simulink model "h16k_ver110_1080"  (R2012b)
settings: Solver=VariableStepDiscrete  SolverMode=SingleTasking  StartTime=0.0  StopTime=128000  RelTol=1e-3
undefined symbols (not defined in the file or in its folder): sfp
libraries: xbsIndex_r4 x3384, dspsigops x32, casper_library_misc x23, monroe_library x8, simulink x7, xps_library x6
(part 1 of 28)
settings Model: Creator=mwagner  LastModifiedBy=ptcs
settings DataIOCC: SignalLoggingSaveFormat=ModelDataLogs
settings OptimizationCC: InlineParams=on
settings DebuggingCC: FcnCallInpInsideContextMsg=UseLocalSettings  StrictBusMsg=Warning
settings GRTTargetCC: CombineOutputUpdateFcns=off  GRTInterface=on

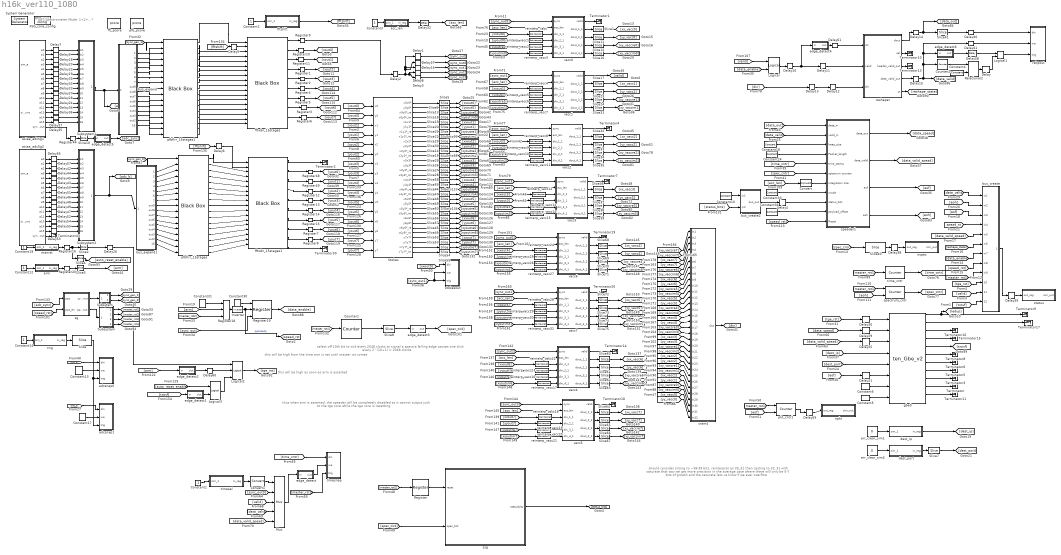
== system h16k_ver110_1080 ==
  note: GBT Spectrometer
      | Mode: 1+2+...?
  note: this will be high from the time arm is set until master rst comes
  note: this will be high as soon as arm is asserted
  note: thus when arm is asserted, the speader will be completely disabled so it cannot output junk to the tge core while the tge core is resetting
  note: should consider slicing to ~38-39 bits, reinterpret as 39_31 then casting to  32_31 with saturate
      | that way we get more precision in the average case where there will only be 5-7 bits of growth
      | and the saturate lets us know if we ever overflow
  note: select off 10th bit to tick every 2048 clocks to signal a spectra
      | falling edge causes one click every 2^(10+1) = 2048 clocks
  " System Generator" : xbsIndex_r4/ System Generator  Tag=genX  xilinxfamily=virtex6  part=xc6vsx475t  speed=-1  package=ff1759  synthesis_tool=XST  clock_wrapper=Clock Enables  directory=./h16k_ver110_1080/sysgen  proj_type=Project Navigator  Synth_file=XST Defaults  Impl_file=ISE Defaults  testbench=off  simulink_period=1  sysclk_period=7.4074  dcm_input_clock_period=100  incr_netlist=off  trim_vbits=Everywhere in SubSystem  dbl_ovrd=According to Block Masks  core_generation=According to Block Masks  run_coregen=off  deprecated_control=off  eval_field=0  block_type=sysgen
      settings: block_version=10.1.3
  Constant{1..3,12,14,19} (6 alike) : Constant
  Constant10 : xbsIndex_r4/Constant  const=0  gui_display_data_type=Fixed-point  arith_type=Unsigned  n_bits=36  bin_pt=0  preci_type=Single  exp_width=8  frac_width=24  explicit_period=on  period=1  equ=P=C  opselect=C  inp2=PCIN>>17  opr=+  inp1=P  carry=CIN  dbl_ovrd=off  block_type=constant
  Constant13 : xbsIndex_r4/Constant  const=1  gui_display_data_type=Boolean  arith_type=Boolean  n_bits=32  bin_pt=0  preci_type=Single  exp_width=8  frac_width=24  explicit_period=on  period=1  equ=P=C  opselect=C  inp2=PCIN>>17  opr=+  inp1=P  carry=CIN  dbl_ovrd=off  block_type=constant
      settings: block_version=11.4
  Constant17 : xbsIndex_r4/Constant  const=1  gui_display_data_type=Boolean  arith_type=Boolean  n_bits=32  bin_pt=0  preci_type=Single  exp_width=8  frac_width=24  explicit_period=on  period=1  equ=P=C  opselect=C  inp2=PCIN>>17  opr=+  inp1=P  carry=CIN  dbl_ovrd=off  block_type=constant
      settings: block_version=11.4
  Constant18 : xbsIndex_r4/Constant  const=262144+8*6  gui_display_data_type=Fixed-point  arith_type=Unsigned  n_bits=40  bin_pt=0  preci_type=Single  exp_width=8  frac_width=24  explicit_period=on  period=1  equ=P=C  opselect=C  inp2=PCIN>>17  opr=+  inp1=P  carry=CIN  dbl_ovrd=off  block_type=constant
  Constant24 : xbsIndex_r4/Constant  const=8192  gui_display_data_type=Fixed-point  arith_type=Unsigned  n_bits=40  bin_pt=0  preci_type=Single  exp_width=8  frac_width=24  explicit_period=on  period=1  equ=P=C  opselect=C  inp2=PCIN>>17  opr=+  inp1=P  carry=CIN  dbl_ovrd=off  block_type=constant
  Constant30 : xbsIndex_r4/Constant  const=1  gui_display_data_type=Fixed-point  arith_type=Boolean  n_bits=16  bin_pt=0  preci_type=Single  exp_width=8  frac_width=24  explicit_period=on  period=1  equ=P=C  opselect=C  inp2=PCIN>>17  opr=+  inp1=P  carry=CIN  dbl_ovrd=off  block_type=constant
      settings: block_version=11.4
  Constant31 : xbsIndex_r4/Constant  const=1  gui_display_data_type=Fixed-point  arith_type=Boolean  n_bits=16  bin_pt=0  preci_type=Single  exp_width=8  frac_width=24  explicit_period=on  period=1  equ=P=C  opselect=C  inp2=PCIN>>17  opr=+  inp1=P  carry=CIN  dbl_ovrd=off  block_type=constant
      settings: block_version=11.4
  Constant33 : xbsIndex_r4/Constant  const=1  gui_display_data_type=Fixed-point  arith_type=Unsigned  n_bits=40  bin_pt=0  preci_type=Single  exp_width=8  frac_width=24  explicit_period=on  period=1  equ=P=C  opselect=C  inp2=PCIN>>17  opr=+  inp1=P  carry=CIN  dbl_ovrd=off  block_type=constant
  Constant34 : xbsIndex_r4/Constant  const=0  gui_display_data_type=Fixed-point  arith_type=Unsigned  n_bits=40  bin_pt=0  preci_type=Single  exp_width=8  frac_width=24  explicit_period=on  period=1  equ=P=C  opselect=C  inp2=PCIN>>17  opr=+  inp1=P  carry=CIN  dbl_ovrd=off  block_type=constant
  Constant4 : xbsIndex_r4/Constant  const=65535  gui_display_data_type=Fixed-point  arith_type=Unsigned  n_bits=16  bin_pt=0  preci_type=Single  exp_width=8  frac_width=24  explicit_period=on  period=1  equ=P=C  opselect=C  inp2=PCIN>>17  opr=+  inp1=P  carry=CIN  dbl_ovrd=off  block_type=constant
  Constant5 : xbsIndex_r4/Constant  const=1  gui_display_data_type=Boolean  arith_type=Boolean  n_bits=1  bin_pt=0  preci_type=Single  exp_width=8  frac_width=24  explicit_period=on  period=1  equ=P=C  opselect=C  inp2=PCIN>>17  opr=+  inp1=P  carry=CIN  dbl_ovrd=off  block_type=constant
  Constant6 : xbsIndex_r4/Constant  const=1  gui_display_data_type=Boolean  arith_type=Boolean  n_bits=1  bin_pt=0  preci_type=Single  exp_width=8  frac_width=24  explicit_period=on  period=1  equ=P=C  opselect=C  inp2=PCIN>>17  opr=+  inp1=P  carry=CIN  dbl_ovrd=off  block_type=constant
  Convert : xbsIndex_r4/Convert  gui_display_data_type=Fixed-point  arith_type=Unsigned  n_bits=40  bin_pt=0  float_type=Single  exp_bits=8  fraction_bits=24  quantization=Truncate  overflow=Wrap  en=off  latency=0  dbl_ovrd=off  pipeline=off  block_type=convert
      settings: block_version=11.4
  Convert1 : xbsIndex_r4/Convert  gui_display_data_type=Fixed-point  arith_type=Unsigned  n_bits=2  bin_pt=0  float_type=Single  exp_bits=8  fraction_bits=24  quantization=Truncate  overflow=Wrap  en=off  latency=1  dbl_ovrd=off  pipeline=off  block_type=convert
  Counter1 : xbsIndex_r4/Counter  cnt_type=Free Running  cnt_to=Inf  operation=Up  start_count=0  cnt_by_val=1  arith_type=Unsigned  n_bits=48  bin_pt=0  load_pin=off  rst=on  en=off  explicit_period=on  period=1  dbl_ovrd=off  use_behavioral_HDL=off  implementation=DSP48  block_type=counter
      settings: block_version=11.3
  Counter2 : xbsIndex_r4/Counter  cnt_type=Free Running  cnt_to=Inf  operation=Down  start_count=65535  cnt_by_val=1  arith_type=Unsigned  n_bits=16  bin_pt=0  load_pin=off  rst=off  en=on  explicit_period=on  period=1  dbl_ovrd=off  use_behavioral_HDL=off  implementation=Fabric  block_type=counter
  Delay{,1,3,5..6,8,16..17,32} (9 alike) : xbsIndex_r4/Delay  rst=off  infoeditControl=Selection of Reset will increase slice count due to use of real FFs and instead of SRLs  en=off  latency=1  dbl_ovrd=off  reg_retiming=off  block_type=delay
      Delay1 settings: block_version=11.4
      Delay16 settings: block_version=11.4
      Delay17 settings: block_version=11.4
      Delay3 settings: block_version=11.4
      Delay32 settings: block_version=11.4
      Delay5 settings: block_version=11.4
      Delay6 settings: block_version=11.4
      Delay8 settings: block_version=11.4
  Delay{10..13,58} (5 alike) : xbsIndex_r4/Delay  rst=off  infoeditControl=Selection of Reset will increase slice count due to use of real FFs and instead of SRLs  en=off  latency=2  dbl_ovrd=off  reg_retiming=off  block_type=delay
  Delay{14..15,40..41} (4 alike) : xbsIndex_r4/Delay  rst=off  infoeditControl=Selection of Reset will increase slice count due to use of real FFs and instead of SRLs  en=off  latency=4  dbl_ovrd=off  reg_retiming=on  block_type=delay
  Delay{4,7,9,18..25,27..31,33..39,42..57,59} (40 alike) : xbsIndex_r4/Delay  rst=off  infoeditControl=Selection of Reset will increase slice count due to use of real FFs and instead of SRLs  en=off  latency=1  dbl_ovrd=off  reg_retiming=on  block_type=delay
      Delay18 settings: block_version=11.4
      Delay19 settings: block_version=11.4
      Delay20 settings: block_version=11.4
      Delay22 settings: block_version=11.4
      Delay23 settings: block_version=11.4
      Delay24 settings: block_version=11.4
      Delay27 settings: block_version=11.4
      Delay28 settings: block_version=11.4
      Delay31 settings: block_version=11.4
      Delay33 settings: block_version=11.4
      Delay34 settings: block_version=11.4
      Delay35 settings: block_version=11.4
      Delay36 settings: block_version=11.4
      Delay37 settings: block_version=11.4
      Delay42 settings: block_version=11.4
      Delay43 settings: block_version=11.4
      Delay44 settings: block_version=11.4
      Delay45 settings: block_version=11.4
      Delay46 settings: block_version=11.4
      Delay47 settings: block_version=11.4
      Delay48 settings: block_version=11.4
      Delay49 settings: block_version=11.4
      Delay50 settings: block_version=11.4
      Delay51 settings: block_version=11.4
      Delay52 settings: block_version=11.4
      Delay53 settings: block_version=11.4
      Delay54 settings: block_version=11.4
      Delay55 settings: block_version=11.4
      Delay56 settings: block_version=11.4
      Delay57 settings: block_version=11.4
      Delay7 settings: block_version=11.4
      Delay9 settings: block_version=11.4
  Delay2 : xbsIndex_r4/Delay  rst=off  infoeditControl=Selection of Reset will increase slice count due to use of real FFs and instead of SRLs  en=off  latency=3  dbl_ovrd=off  reg_retiming=off  block_type=delay
      settings: block_version=11.4
  Delay26 : xbsIndex_r4/Delay  rst=off  infoeditControl=Selection of Reset will increase slice count due to use of real FFs and instead of SRLs  en=off  latency=8  dbl_ovrd=off  reg_retiming=on  block_type=delay
  Delay60 : xbsIndex_r4/Delay  rst=off  infoeditControl=Selection of Reset will increase slice count due to use of real FFs and instead of SRLs  en=off  latency=16  dbl_ovrd=off  reg_retiming=off  block_type=delay
      settings: block_version=11.4
  Delay61 : xbsIndex_r4/Delay  rst=off  infoeditControl=Selection of Reset will increase slice count due to use of real FFs and instead of SRLs  en=off  latency=10  dbl_ovrd=off  reg_retiming=off  block_type=delay
  Inverter : xbsIndex_r4/Inverter  en=off  latency=0  dbl_ovrd=off  block_type=inv
      settings: block_version=11.4
  Logical : xbsIndex_r4/Logical  logical_function=AND  inputs=2  en=off  latency=0  precision=Full  arith_type=Unsigned  n_bits=16  bin_pt=0  align_bp=on  dbl_ovrd=off  block_type=logical
      settings: block_version=11.4
  Logical1 : xbsIndex_r4/Logical  logical_function=AND  inputs=2  en=off  latency=1  precision=Full  arith_type=Unsigned  n_bits=16  bin_pt=0  align_bp=on  dbl_ovrd=off  block_type=logical
  Logical2 : xbsIndex_r4/Logical  logical_function=OR  inputs=3  en=off  latency=0  precision=Full  arith_type=Unsigned  n_bits=8  bin_pt=2  align_bp=on  dbl_ovrd=off  block_type=logical
      settings: xl_area=[0, 0, 0, 0, 0, 0, 0]
  Logical3 : xbsIndex_r4/Logical  logical_function=AND  inputs=2  en=off  latency=1  precision=Full  arith_type=Unsigned  n_bits=8  bin_pt=2  align_bp=on  dbl_ovrd=off  block_type=logical
      settings: xl_area=[0, 0, 0, 0, 0, 0, 0]
  Mux : xbsIndex_r4/Mux  inputs=4  en=off  latency=1  precision=Full  arith_type=Unsigned  n_bits=16  bin_pt=14  quantization=Truncate  overflow=Wrap  dbl_ovrd=off  block_type=mux
  Register{,1..16,20,44,48..49} (21 alike) : xbsIndex_r4/Register  init=0  rst=off  en=off  dbl_ovrd=off  block_type=register
      settings: block_version=11.4
  Register18 : xbsIndex_r4/Register  init=0  rst=on  en=on  dbl_ovrd=off  block_type=register
      settings: block_version=11.4
  Register19 : xbsIndex_r4/Register  init=0  rst=on  en=on  dbl_ovrd=off  block_type=register
      settings: block_version=11.4
  Relational2 : xbsIndex_r4/Relational  mode=a=b  en=off  latency=1  dbl_ovrd=off  block_type=relational
  Slice{,2..3,10} (4 alike) : xbsIndex_r4/Slice  nbits=1  boolean_output=on  mode=Lower Bit Location + Width  bit1=0  base1=MSB of Input  bit0=0  base0=LSB of Input  dbl_ovrd=off  block_type=slice
      Slice10 settings: infoedit="Extracts a given range of bits from each input sample and presents it at the output.  The output type is ordinarily unsigned with binary point at zero, but can be Boolean when the slice is one bit wide.<P><P>Hardware notes: In hardware this block costs nothing."  block_version=10.1.3
      Slice2 settings: block_version=10.1.3
      Slice3 settings: block_version=10.1.3
  Slice{1,5..6,11..39,41,44..75} (65 alike) : xbsIndex_r4/Slice  nbits=32  boolean_output=off  mode=Upper Bit Location + Width  bit1=0  base1=MSB of Input  bit0=0  base0=LSB of Input  dbl_ovrd=off  block_type=slice
  Slice4 : xbsIndex_r4/Slice  nbits=1  boolean_output=on  mode=Lower Bit Location + Width  bit1=0  base1=MSB of Input  bit0=1  base0=LSB of Input  dbl_ovrd=off  block_type=slice
      settings: block_version=10.1.3
  Slice40 : xbsIndex_r4/Slice  nbits=32  boolean_output=off  mode=Lower Bit Location + Width  bit1=0  base1=MSB of Input  bit0=0  base0=LSB of Input  dbl_ovrd=off  block_type=slice
  Slice7 : xbsIndex_r4/Slice  nbits=16  boolean_output=off  mode=Lower Bit Location + Width  bit1=0  base1=MSB of Input  bit0=0  base0=LSB of Input  dbl_ovrd=off  block_type=slice
      settings: infoedit="Extracts a given range of bits from each input sample and presents it at the output.  The output type is ordinarily unsigned with binary point at zero, but can be Boolean when the slice is one bit wide.<P><P>Hardware notes: In hardware this block costs nothing."  block_version=10.1.3
  Slice8 : xbsIndex_r4/Slice  nbits=1  boolean_output=on  mode=Lower Bit Location + Width  bit1=7  base1=MSB of Input  bit0=10  base0=LSB of Input  dbl_ovrd=off  block_type=slice
      settings: block_version=10.1.3
  Stokes : Subsystem  mask{n_samples=8, addlatency=2}
      mask prompts: n_samples "Number of simultaneous inputs"; addlatency "Adder latency"
      mask init:
      | % To make the xBlock smart so it won''t re-generate the
      | % subsystem if neither the arguments nor the scripts are
      | % changes, use as the following:
      | cfg.source = str2func('stokes_init');
      | cfg.toplevel = gcb;
      | cfg.depend = {'stokes_init'};
      | args = {n_samples, addlatency};
      | xBlock(cfg, args);
  Subsystem : Subsystem
  Subsystem1 : Subsystem
  Subsystem2 : Subsystem
  Subsytem : Subsystem
  Terminator{,1..11,13..20,30,43} (22 alike) : Terminator
  XSG_core_config : xps_library/XSG core config  Tag=xps:xsg  hw_sys=ROACH2:sx475t  clk_src=adc0_clk  ROACH_clk_src=adc0_clk  ROACH2_clk_src=adc0_clk  MKDIG_clk_src=sys_clk  clk_rate=135  sample_period=1  synthesis_tool=XST
  acc_len : Subsystem  Tag=xps:sw_reg  AncestorBlock=xps_library/software register  mask(swreg){mode=one value, io_dir=From Processor, io_delay=0, sample_period=1, names=reg, bitwidths=32, arith_types=0, bin_pts=0, sim_port=on, show_format=off}
      mask prompts: io_dir "I/O direction"; io_delay "I/O delay"; sample_period "Sample period"; names "Name:"; bitwidths "Bitwidth:"; arith_types "Type (ufix=0, fix=1, bool=2):"; bin_pts "Binary pt:"; sim_port "Provide sim input/output?"; show_format "Print format string?"
      mask init:
      | swreg_init(gcb)
      settings: AttributesFormatString=1input
      mask TypeOptions mode: one value | fields of equal size | fields of arbitrary size
      mask Callback mode: swreg_cb(gcb);
      mask TypeOptions io_dir: To Processor | From Processor
      mask Callback io_dir:
      | mask_enables = get_param(gcb, 'MaskEnables');
      | mask_names = get_param(gcb, 'MaskNames');
      | if strcmp(get_param(gcb, 'io_dir'), 'To Processor'),
      |     mask_enables{ismember(mask_names, 'sample_period')} = 'off';
      | else
      |     mask_enables{ismember(mask_names, 'sample_period')} = 'on';
      | end
      | set_param(gcb, 'MaskEnables', mask_enables);
      mask Callback bitwidths:
      | swreg_maskcheck(gcb);
      | % blk = gcb;
      | % mode = get_param(blk, 'mode');
      | % current_widths = eval(get_param(blk, 'bitwidths'));
      | % if (strcmp(mode, 'one value') || strcmp(mode, 'fields of equal size')) && (length(current_widths) > 1),
      | %     error('Only one width may be specified for this mode.');
      | % elseif strcmp(mode, 'fields of arbitrary size')
      | %     current_names = textscan(strtrim(strrep(strrep(get_param(blk, 'names'), ']', ''), '[', '')), '%s');
      | %     current_names = current_names{1};
      | %     numios = length(current_names);
      | %     if length(current_widths) ~= numios,
      | %         error('%d field names specified, but %d widths?', numios, length(current_widths));
      | %     end
      | % end
      | % total_width = 0;
      | % for ctr = 1 : length(current_widths),
      | %     total_width = total_width + current_widths(ctr);
      | % end
      | % if total_width > 32,
      | %     error('Total width must be 32 or less, set to %d.', total_width);
      | % end
      mask Callback arith_types:
      | [numios, ~, ~, ~, current_types] = swreg_maskcheck(gcb);
      | % blk = gcb;
      | % mode = get_param(blk, 'mode');
      | % current_types = eval(get_param(blk, 'arith_types'));
      | % numios = length(current_types);
      | % if (strcmp(mode, 'one value') || strcmp(mode, 'fields of equal size')) && (length(current_types) > 1),
      | %     error('Only one type may be specified for this mode.');
      | % elseif strcmp(mode, 'fields of arbitrary size')
      | %     current_names = textscan(strtrim(strrep(strrep(get_param(blk, 'names'), ']', ''), '[', '')), '%s');
      | %     current_names = current_names{1};
      | %     numios = length(current_names);
      | %     if length(current_types) ~= numios,
      | %         error('%d field names specified, but %d types?', numios, length(current_types));
      | %     end
      | % end
      | problem = 0;
      | for ctr = 1 : numios,
      |     t = current_types(ctr);
      |     if (t < 0) || (t > 2),
      |         problem = t;
      |         ctr = numios + 1;
      |     end
      | end
      | if problem ~= 0,
      |     error('Type cannot be %i, must be 0, 1 or 2.', problem);
      | end
      mask Callback bin_pts:
      | swreg_maskcheck(gcb);
      | % blk = gcb;
      | % mode = get_param(blk, 'mode');
      | % current_bins = eval(get_param(blk, 'bin_pts'));
      | % if (strcmp(mode, 'one value') || strcmp(mode, 'fields of equal size')) && (length(current_bins) > 1),
      | %     error('Only one binary pt may be specified for this mode.');
      | % elseif strcmp(mode, 'fields of arbitrary size')
      | %     current_names = textscan(strtrim(strrep(strrep(get_param(blk, 'names'), ']', ''), '[', '')), '%s');
      | %     current_names = current_names{1};
      | %     numios = length(current_names);
      | %     if length(current_bins) ~= numios,
      | %         error('%d field names specified, but %d binary pts?', numios, length(current_bins));
      | %     end
      | % end
  adcsnap0 : Subsystem  Tag=casper:snapshot  AncestorBlock=casper_library_scopes/snapshot  mask(snapshot){storage=bram, dram_dimm=1, dram_clock=200, nsamples=10, data_width=128, offset=off, circap=off, value=off, use_dsp48=on}
      mask prompts: storage "Storage medium"; dram_dimm "DRAM dimm"; dram_clock "DRAM clock rate"; nsamples "Number of Samples (2^?)"; data_width "Data width"; offset "Start delay support"; circap "Circular capture support"; value "Extra value capture support"; use_dsp48 "Use DSP48s to implement counters"
      mask help:
      | Standard snap block, but with the following optional extras;
      |  1) Optionally delay the fabric trigger by a user-specified number of valids.
      |  2) Capture continuously after a trigger until a stop pulse is received. Data is captured into BRAM continuously, with old data being overwritten until a stop command is received. Then stop capturing when memory is filled. This enables you to get some data before and some data after the stop pulse. Use the 'tr_en_cnt' register to determine where you are in your vector. 'Addr' register's MSb now indicates 'busy capturing'.
      |  3) Optionally capture a value on an input port to a register at the same time as the first data sample.
      |  4) Implement counters using DSP48Es to save resources.
      mask init:
      | snapshot_init(gcb, ...
      |     'storage', storage, ...
      |     'dram_dimm', dram_dimm, ...
      |     'dram_clock', dram_clock, ...
      |     'nsamples', nsamples, ...
      |     'data_width', data_width, ...
      |     'offset', offset, ...
      |     'circap', circap, ...
      |     'value', value, ...
      |     'use_dsp48', use_dsp48);
      mask TypeOptions storage: bram | dram
      mask Callback storage: snapshot_callback();
      mask TypeOptions dram_dimm: 1 | 2 | 3 | 4
      mask TypeOptions dram_clock: 200 | 250 | 266 | 300 | 333
      mask TypeOptions data_width: 8 | 16 | 32 | 64 | 128
  adcsnap1 : Subsystem  Tag=casper:snapshot  AncestorBlock=casper_library_scopes/snapshot  mask(snapshot){storage=bram, dram_dimm=1, dram_clock=200, nsamples=10, data_width=128, offset=off, circap=off, value=off, use_dsp48=on}
      mask prompts: storage "Storage medium"; dram_dimm "DRAM dimm"; dram_clock "DRAM clock rate"; nsamples "Number of Samples (2^?)"; data_width "Data width"; offset "Start delay support"; circap "Circular capture support"; value "Extra value capture support"; use_dsp48 "Use DSP48s to implement counters"
      mask help:
      | Standard snap block, but with the following optional extras;
      |  1) Optionally delay the fabric trigger by a user-specified number of valids.
      |  2) Capture continuously after a trigger until a stop pulse is received. Data is captured into BRAM continuously, with old data being overwritten until a stop command is received. Then stop capturing when memory is filled. This enables you to get some data before and some data after the stop pulse. Use the 'tr_en_cnt' register to determine where you are in your vector. 'Addr' register's MSb now indicates 'busy capturing'.
      |  3) Optionally capture a value on an input port to a register at the same time as the first data sample.
      |  4) Implement counters using DSP48Es to save resources.
      mask init: same as h16k_ver110_1080/adcsnap0
      mask TypeOptions storage: bram | dram
      mask Callback storage: snapshot_callback();
      mask TypeOptions dram_dimm: 1 | 2 | 3 | 4
      mask TypeOptions dram_clock: 200 | 250 | 266 | 300 | 333
      mask TypeOptions data_width: 8 | 16 | 32 | 64 | 128
  arm : Subsystem  Tag=xps:sw_reg  AncestorBlock=xps_library/software register  mask(swreg){mode=one value, io_dir=From Processor, io_delay=0, sample_period=1, names=reg, bitwidths=32, arith_types=0, bin_pts=0, sim_port=on, show_format=off}
      mask prompts: io_dir "I/O direction"; io_delay "I/O delay"; sample_period "Sample period"; names "Name:"; bitwidths "Bitwidth:"; arith_types "Type (ufix=0, fix=1, bool=2):"; bin_pts "Binary pt:"; sim_port "Provide sim input/output?"; show_format "Print format string?"
      mask init:
      | swreg_init(gcb)
      settings: AttributesFormatString=1input
      mask TypeOptions mode: one value | fields of equal size | fields of arbitrary size
      mask Callback mode: swreg_cb(gcb);
      mask TypeOptions io_dir: To Processor | From Processor
      mask Callback io_dir:
      | mask_enables = get_param(gcb, 'MaskEnables');
      | mask_names = get_param(gcb, 'MaskNames');
      | if strcmp(get_param(gcb, 'io_dir'), 'To Processor'),
      |     mask_enables{ismember(mask_names, 'sample_period')} = 'off';
      | else
      |     mask_enables{ismember(mask_names, 'sample_period')} = 'on';
      | end
      | set_param(gcb, 'MaskEnables', mask_enables);
      mask Callback bitwidths:
      | swreg_maskcheck(gcb);
      | % blk = gcb;
      | % mode = get_param(blk, 'mode');
      | % current_widths = eval(get_param(blk, 'bitwidths'));
      | % if (strcmp(mode, 'one value') || strcmp(mode, 'fields of equal size')) && (length(current_widths) > 1),
      | %     error('Only one width may be specified for this mode.');
      | % elseif strcmp(mode, 'fields of arbitrary size')
      | %     current_names = textscan(strtrim(strrep(strrep(get_param(blk, 'names'), ']', ''), '[', '')), '%s');
      | %     current_names = current_names{1};
      | %     numios = length(current_names);
      | %     if length(current_widths) ~= numios,
      | %         error('%d field names specified, but %d widths?', numios, length(current_widths));
      | %     end
      | % end
      | % total_width = 0;
      | % for ctr = 1 : length(current_widths),
      | %     total_width = total_width + current_widths(ctr);
      | % end
      | % if total_width > 32,
      | %     error('Total width must be 32 or less, set to %d.', total_width);
      | % end
      mask Callback arith_types:
      | [numios, ~, ~, ~, current_types] = swreg_maskcheck(gcb);
      | % blk = gcb;
      | % mode = get_param(blk, 'mode');
      | % current_types = eval(get_param(blk, 'arith_types'));
      | % numios = length(current_types);
      | % if (strcmp(mode, 'one value') || strcmp(mode, 'fields of equal size')) && (length(current_types) > 1),
      | %     error('Only one type may be specified for this mode.');
      | % elseif strcmp(mode, 'fields of arbitrary size')
      | %     current_names = textscan(strtrim(strrep(strrep(get_param(blk, 'names'), ']', ''), '[', '')), '%s');
      | %     current_names = current_names{1};
      | %     numios = length(current_names);
      | %     if length(current_types) ~= numios,
      | %         error('%d field names specified, but %d types?', numios, length(current_types));
      | %     end
      | % end
      | problem = 0;
      | for ctr = 1 : numios,
      |     t = current_types(ctr);
      |     if (t < 0) || (t > 2),
      |         problem = t;
      |         ctr = numios + 1;
      |     end
      | end
      | if problem ~= 0,
      |     error('Type cannot be %i, must be 0, 1 or 2.', problem);
      | end
      mask Callback bin_pts:
      | swreg_maskcheck(gcb);
      | % blk = gcb;
      | % mode = get_param(blk, 'mode');
      | % current_bins = eval(get_param(blk, 'bin_pts'));
      | % if (strcmp(mode, 'one value') || strcmp(mode, 'fields of equal size')) && (length(current_bins) > 1),
      | %     error('Only one binary pt may be specified for this mode.');
      | % elseif strcmp(mode, 'fields of arbitrary size')
      | %     current_names = textscan(strtrim(strrep(strrep(get_param(blk, 'names'), ']', ''), '[', '')), '%s');
      | %     current_names = current_names{1};
      | %     numios = length(current_names);
      | %     if length(current_bins) ~= numios,
      | %         error('%d field names specified, but %d binary pts?', numios, length(current_bins));
      | %     end
      | % end
  asiaa_adc5g1 : Subsystem  Tag=xps:adc5g  AncestorBlock=xps_library/ADCs/asiaa_adc5g  mask(adc5g){input_mode=One-channel -- A, adc_brd=ZDOK 0, demux=1:1, adc_bit_width=8, adc_clk_rate=1080, using_ctrl=on, test_ramp=off}
      mask prompts: input_mode "Input mode:"; adc_brd "ADC Board"; demux "Internal demux"; adc_bit_width "ADC Resolution (bits):"; adc_clk_rate "ADC Clock Rate (MHz):"; using_ctrl "use control"; test_ramp "start in test ramp mode"
      mask help:
      | Interface for the ASIAA 5 GSps ADC. Supports interleaving all four
      | cores using either input A or C, or interleaving two-cores each for
      | A and C. The hardware itself comes in two versions:
      |
      | DMUX 1:2 -- 4-bit samples, 4 parallel streams
      | DMUX 1:1 -- 8-bit samples, 2 parallel streams
      |
      | In either configuration this block will output 8 parallel streams
      | but the underlying interface, and the bitwidth of the samples,
      | will be different.
      mask init:
      | adc5g_init(gcb,...
      |     'input_mode', input_mode,...
      |     'demux', demux,...
      |     'adc_clk_rate', adc_clk_rate,...
      |     'adc_bit_width', adc_bit_width,...
      |     'adc_brd', adc_brd,...
      |     'using_ctrl', using_ctrl,...
      |     'test_ramp', test_ramp);
      mask TypeOptions input_mode: One-channel -- A | One-channel -- C | Two-channel -- A&C
      mask TypeOptions adc_brd: ZDOK 0 | ZDOK 1
      mask TypeOptions demux: 1:1 | 1:2
      mask Callback demux:
      | demux = get_param(gcb,'demux');
      | if(strcmp(demux,'1:1')),
      |     set_param(gcb, 'adc_bit_width', '8')
      | elseif(strcmp(demux, '1:2')),
      |     set_param(gcb, 'adc_bit_width', '4');
      | else
      | end
  asiaa_adc5g2 : Subsystem  Tag=xps:adc5g  AncestorBlock=xps_library/ADCs/asiaa_adc5g  mask(adc5g){input_mode=One-channel -- A, adc_brd=ZDOK 1, demux=1:1, adc_bit_width=8, adc_clk_rate=1080, using_ctrl=on, test_ramp=off}
      mask prompts: input_mode "Input mode:"; adc_brd "ADC Board"; demux "Internal demux"; adc_bit_width "ADC Resolution (bits):"; adc_clk_rate "ADC Clock Rate (MHz):"; using_ctrl "use control"; test_ramp "start in test ramp mode"
      mask help:
      | Interface for the ASIAA 5 GSps ADC. Supports interleaving all four
      | cores using either input A or C, or interleaving two-cores each for
      | A and C. The hardware itself comes in two versions:
      |
      | DMUX 1:2 -- 4-bit samples, 4 parallel streams
      | DMUX 1:1 -- 8-bit samples, 2 parallel streams
      |
      | In either configuration this block will output 8 parallel streams
      | but the underlying interface, and the bitwidth of the samples,
      | will be different.
      mask init: same as h16k_ver110_1080/asiaa_adc5g1
      mask TypeOptions input_mode: One-channel -- A | One-channel -- C | Two-channel -- A&C
      mask TypeOptions adc_brd: ZDOK 0 | ZDOK 1
      mask TypeOptions demux: 1:1 | 1:2
      mask Callback demux:
      | demux = get_param(gcb,'demux');
      | if(strcmp(demux,'1:1')),
      |     set_param(gcb, 'adc_bit_width', '8')
      | elseif(strcmp(demux, '1:2')),
      |     set_param(gcb, 'adc_bit_width', '4');
      | else
      | end
  bus_create : Subsystem  AncestorBlock=casper_library_flow_control/bus_create  mask(bus_create){inputNum=12}
      mask prompts: inputNum "Number of inputs:"
      mask init:
      | bus_create_init(gcb,...
      |     'inputNum', inputNum);
  bus_create2 : Subsystem  AncestorBlock=casper_library_flow_control/bus_create  mask(bus_create){inputNum=2}
      mask prompts: inputNum "Number of inputs:"
      mask init:
      | bus_create_init(gcb,...
      |     'inputNum', inputNum);
  bus_expand : Subsystem  AncestorBlock=casper_library_flow_control/bus_expand  mask(bus_expand){mode=divisions of equal size, outputNum=16, outputWidth=8, outputBinaryPt=7, outputArithmeticType=1, show_format=off, outputToWorkspace=off, variablePrefix=out, outputToModelAsWell=on}
      mask prompts: outputNum "Number of outputs:"; outputWidth "Output width:"; outputBinaryPt "Output binary point position:"; outputArithmeticType "Output arithmetic type (ufix=0, fix=1, bool=2):"; show_format "Print format string?"; outputToWorkspace "Output to workspace?"; variablePrefix "Variable name prefix:"; outputToModelAsWell "Output to model as well?"
      mask help:
      | Expands a 'bus' made using a bus_create or Xilinx
      | concat block.
      | The input will be divided into the specified number
      | of outputs with the specified arithmetic types.
      | Divisions are made from most significant bit.
      mask init:
      | bus_expand_init(gcb,...
      |     'mode', mode, ...
      |     'outputNum', outputNum, ...
      |     'outputWidth', outputWidth, ...
      |     'outputBinaryPt', outputBinaryPt, ...
      |     'outputArithmeticType', outputArithmeticType, ...
      |     'show_format', show_format, ...
      |     'outputToWorkspace', outputToWorkspace, ...
      |     'variablePrefix', variablePrefix, ...
      |     'outputToModelAsWell', outputToModelAsWell);
      settings: AttributesFormatString=16 outputs
      mask TypeOptions mode: divisions of equal size | divisions of arbitrary size
      mask Callback mode: bus_expand_callback();
      mask Callback outputWidth: bus_expand_callback();
      mask Callback outputToWorkspace: bus_expand_callback();
  bus_expand1 : Subsystem  AncestorBlock=casper_library_flow_control/bus_expand  mask(bus_expand){mode=divisions of equal size, outputNum=16, outputWidth=8, outputBinaryPt=7, outputArithmeticType=1, show_format=off, outputToWorkspace=off, variablePrefix=out, outputToModelAsWell=on}
      mask prompts: outputNum "Number of outputs:"; outputWidth "Output width:"; outputBinaryPt "Output binary point position:"; outputArithmeticType "Output arithmetic type (ufix=0, fix=1, bool=2):"; show_format "Print format string?"; outputToWorkspace "Output to workspace?"; variablePrefix "Variable name prefix:"; outputToModelAsWell "Output to model as well?"
      mask help:
      | Expands a 'bus' made using a bus_create or Xilinx
      | concat block.
      | The input will be divided into the specified number
      | of outputs with the specified arithmetic types.
      | Divisions are made from most significant bit.
      mask init: same as h16k_ver110_1080/bus_expand
      settings: AttributesFormatString=16 outputs
      mask TypeOptions mode: divisions of equal size | divisions of arbitrary size
      mask Callback mode: bus_expand_callback();
      mask Callback outputWidth: bus_expand_callback();
      mask Callback outputToWorkspace: bus_expand_callback();
  cram4 : Subsystem  AncestorBlock=gavrt_library/cram  mask(cram){num_slice=32}
      mask prompts: num_slice "Number of slices"
      mask help: Concatenates inputs together after forcing binary point to zero.
      mask init:
      | cram_init(gcb, ...
      |     'num_slice', num_slice);
  dest_ip : Subsystem  Tag=xps:sw_reg  AncestorBlock=xps_library/software register  mask(swreg){mode=one value, io_dir=From Processor, io_delay=0, sample_period=1, names=reg, bitwidths=32, arith_types=0, bin_pts=0, sim_port=on, show_format=off}
      mask prompts: io_dir "I/O direction"; io_delay "I/O delay"; sample_period "Sample period"; names "Name:"; bitwidths "Bitwidth:"; arith_types "Type (ufix=0, fix=1, bool=2):"; bin_pts "Binary pt:"; sim_port "Provide sim input/output?"; show_format "Print format string?"
      mask init:
      | swreg_init(gcb)
      settings: AttributesFormatString=1input
      mask TypeOptions mode: one value | fields of equal size | fields of arbitrary size
      mask Callback mode: swreg_cb(gcb);
      mask TypeOptions io_dir: To Processor | From Processor
      mask Callback io_dir:
      | mask_enables = get_param(gcb, 'MaskEnables');
      | mask_names = get_param(gcb, 'MaskNames');
      | if strcmp(get_param(gcb, 'io_dir'), 'To Processor'),
      |     mask_enables{ismember(mask_names, 'sample_period')} = 'off';
      | else
      |     mask_enables{ismember(mask_names, 'sample_period')} = 'on';
      | end
      | set_param(gcb, 'MaskEnables', mask_enables);
      mask Callback bitwidths:
      | swreg_maskcheck(gcb);
      | % blk = gcb;
      | % mode = get_param(blk, 'mode');
      | % current_widths = eval(get_param(blk, 'bitwidths'));
      | % if (strcmp(mode, 'one value') || strcmp(mode, 'fields of equal size')) && (length(current_widths) > 1),
      | %     error('Only one width may be specified for this mode.');
      | % elseif strcmp(mode, 'fields of arbitrary size')
      | %     current_names = textscan(strtrim(strrep(strrep(get_param(blk, 'names'), ']', ''), '[', '')), '%s');
      | %     current_names = current_names{1};
      | %     numios = length(current_names);
      | %     if length(current_widths) ~= numios,
      | %         error('%d field names specified, but %d widths?', numios, length(current_widths));
      | %     end
      | % end
      | % total_width = 0;
      | % for ctr = 1 : length(current_widths),
      | %     total_width = total_width + current_widths(ctr);
      | % end
      | % if total_width > 32,
      | %     error('Total width must be 32 or less, set to %d.', total_width);
      | % end
      mask Callback arith_types:
      | [numios, ~, ~, ~, current_types] = swreg_maskcheck(gcb);
      | % blk = gcb;
      | % mode = get_param(blk, 'mode');
      | % current_types = eval(get_param(blk, 'arith_types'));
      | % numios = length(current_types);
      | % if (strcmp(mode, 'one value') || strcmp(mode, 'fields of equal size')) && (length(current_types) > 1),
      | %     error('Only one type may be specified for this mode.');
      | % elseif strcmp(mode, 'fields of arbitrary size')
      | %     current_names = textscan(strtrim(strrep(strrep(get_param(blk, 'names'), ']', ''), '[', '')), '%s');
      | %     current_names = current_names{1};
      | %     numios = length(current_names);
      | %     if length(current_types) ~= numios,
      | %         error('%d field names specified, but %d types?', numios, length(current_types));
      | %     end
      | % end
      | problem = 0;
      | for ctr = 1 : numios,
      |     t = current_types(ctr);
      |     if (t < 0) || (t > 2),
      |         problem = t;
      |         ctr = numios + 1;
      |     end
      | end
      | if problem ~= 0,
      |     error('Type cannot be %i, must be 0, 1 or 2.', problem);
      | end
      mask Callback bin_pts:
      | swreg_maskcheck(gcb);
      | % blk = gcb;
      | % mode = get_param(blk, 'mode');
      | % current_bins = eval(get_param(blk, 'bin_pts'));
      | % if (strcmp(mode, 'one value') || strcmp(mode, 'fields of equal size')) && (length(current_bins) > 1),
      | %     error('Only one binary pt may be specified for this mode.');
      | % elseif strcmp(mode, 'fields of arbitrary size')
      | %     current_names = textscan(strtrim(strrep(strrep(get_param(blk, 'names'), ']', ''), '[', '')), '%s');
      | %     current_names = current_names{1};
      | %     numios = length(current_names);
      | %     if length(current_bins) ~= numios,
      | %         error('%d field names specified, but %d binary pts?', numios, length(current_bins));
      | %     end
      | % end
  dest_port : Subsystem  Tag=xps:sw_reg  AncestorBlock=xps_library/software register  mask(swreg){mode=one value, io_dir=From Processor, io_delay=0, sample_period=1, names=reg, bitwidths=32, arith_types=0, bin_pts=0, sim_port=on, show_format=off}
      mask prompts: io_dir "I/O direction"; io_delay "I/O delay"; sample_period "Sample period"; names "Name:"; bitwidths "Bitwidth:"; arith_types "Type (ufix=0, fix=1, bool=2):"; bin_pts "Binary pt:"; sim_port "Provide sim input/output?"; show_format "Print format string?"
      mask init:
      | swreg_init(gcb)
      settings: AttributesFormatString=1input
      mask TypeOptions mode: one value | fields of equal size | fields of arbitrary size
      mask Callback mode: swreg_cb(gcb);
      mask TypeOptions io_dir: To Processor | From Processor
      mask Callback io_dir:
      | mask_enables = get_param(gcb, 'MaskEnables');
      | mask_names = get_param(gcb, 'MaskNames');
      | if strcmp(get_param(gcb, 'io_dir'), 'To Processor'),
      |     mask_enables{ismember(mask_names, 'sample_period')} = 'off';
      | else
      |     mask_enables{ismember(mask_names, 'sample_period')} = 'on';
      | end
      | set_param(gcb, 'MaskEnables', mask_enables);
      mask Callback bitwidths:
      | swreg_maskcheck(gcb);
      | % blk = gcb;
      | % mode = get_param(blk, 'mode');
      | % current_widths = eval(get_param(blk, 'bitwidths'));
      | % if (strcmp(mode, 'one value') || strcmp(mode, 'fields of equal size')) && (length(current_widths) > 1),
      | %     error('Only one width may be specified for this mode.');
      | % elseif strcmp(mode, 'fields of arbitrary size')
      | %     current_names = textscan(strtrim(strrep(strrep(get_param(blk, 'names'), ']', ''), '[', '')), '%s');
      | %     current_names = current_names{1};
      | %     numios = length(current_names);
      | %     if length(current_widths) ~= numios,
      | %         error('%d field names specified, but %d widths?', numios, length(current_widths));
      | %     end
      | % end
      | % total_width = 0;
      | % for ctr = 1 : length(current_widths),
      | %     total_width = total_width + current_widths(ctr);
      | % end
      | % if total_width > 32,
      | %     error('Total width must be 32 or less, set to %d.', total_width);
      | % end
      mask Callback arith_types:
      | [numios, ~, ~, ~, current_types] = swreg_maskcheck(gcb);
      | % blk = gcb;
      | % mode = get_param(blk, 'mode');
      | % current_types = eval(get_param(blk, 'arith_types'));
      | % numios = length(current_types);
      | % if (strcmp(mode, 'one value') || strcmp(mode, 'fields of equal size')) && (length(current_types) > 1),
      | %     error('Only one type may be specified for this mode.');
      | % elseif strcmp(mode, 'fields of arbitrary size')
      | %     current_names = textscan(strtrim(strrep(strrep(get_param(blk, 'names'), ']', ''), '[', '')), '%s');
      | %     current_names = current_names{1};
      | %     numios = length(current_names);
      | %     if length(current_types) ~= numios,
      | %         error('%d field names specified, but %d types?', numios, length(current_types));
      | %     end
      | % end
      | problem = 0;
      | for ctr = 1 : numios,
      |     t = current_types(ctr);
      |     if (t < 0) || (t > 2),
      |         problem = t;
      |         ctr = numios + 1;
      |     end
      | end
      | if problem ~= 0,
      |     error('Type cannot be %i, must be 0, 1 or 2.', problem);
      | end
      mask Callback bin_pts:
      | swreg_maskcheck(gcb);
      | % blk = gcb;
      | % mode = get_param(blk, 'mode');
      | % current_bins = eval(get_param(blk, 'bin_pts'));
      | % if (strcmp(mode, 'one value') || strcmp(mode, 'fields of equal size')) && (length(current_bins) > 1),
      | %     error('Only one binary pt may be specified for this mode.');
      | % elseif strcmp(mode, 'fields of arbitrary size')
      | %     current_names = textscan(strtrim(strrep(strrep(get_param(blk, 'names'), ']', ''), '[', '')), '%s');
      | %     current_names = current_names{1};
      | %     numios = length(current_names);
      | %     if length(current_bins) ~= numios,
      | %         error('%d field names specified, but %d binary pts?', numios, length(current_bins));
      | %     end
      | % end
  edge_detect : Subsystem  AncestorBlock=casper_library_misc/edge_detect  mask(edge_detect){edge=Rising, polarity=Active High, x_in=[0 0.08 0.08 0.16 0.16 0.24 0.24 0.32 0.32 0.4], y_in=[-1 -1  1  1  1  1  1  1  1  1], x_out=[0.6 0.68 0.68 0.76 0.76 0.84 0.84 0.92 0.92 1], y_out=[-1 -1  1  1 -1 -1 -1 -1 -1 -1]}
      mask prompts: edge "Edge Type"; polarity "Output Polarity"; x_in "Input X Positions"; y_in "Input Y Positions"; x_out "Output X Positions"; y_out "Output Y Positions"
      mask help: Output is active for one-cycle after each edge of the specified type (i.e. rising, falling or both).
      mask init:
      | edge_detect_init(gcb,...
      |     'edge',edge,...
      |     'polarity',polarity,...
      |     'x_in',x_in,...
      |     'x_out',x_out,...
      |     'y_in',y_in,...
      |     'y_out',y_out);
      | 
      | x_in_num=str2num(getfield(getfield(get_param(gcb,'UserData'),'parameters'),'x_in'));
      | x_out_num=str2num(getfield(getfield(get_param(gcb,'UserData'),'parameters'),'x_out'));
      | y_in_num=str2num(getfield(getfield(get_param(gcb,'UserData'),'parameters'),'y_in'));
      | y_out_num=str2num(getfield(getfield(get_param(gcb,'UserData'),'parameters'),'y_out'));
      settings: AttributesFormatString=|
      | rising edges
      | active high
      mask Help: Output is active for one-cycle after each edge of the specified type (i.e. rising, falling, or both).  Latency is zero.
      mask TypeOptions edge: Rising | Falling | Both
      mask TypeOptions polarity: Active High | Active Low
      mask Display:
      | plot(x_in_num,0.5+y_in_num*0.2);
      | plot(x_out_num,0.5+y_out_num*0.2);
  edge_detect1 : Subsystem  AncestorBlock=casper_library_misc/edge_detect  mask(edge_detect){edge=Rising, polarity=Active High, x_in=[0 0.08 0.08 0.16 0.16 0.24 0.24 0.32 0.32 0.4], y_in=[-1 -1  1  1  1  1  1  1  1  1], x_out=[0.6 0.68 0.68 0.76 0.76 0.84 0.84 0.92 0.92 1], y_out=[-1 -1  1  1 -1 -1 -1 -1 -1 -1]}
      mask prompts: edge "Edge Type"; polarity "Output Polarity"; x_in "Input X Positions"; y_in "Input Y Positions"; x_out "Output X Positions"; y_out "Output Y Positions"
      mask help: Output is active for one-cycle after each edge of the specified type (i.e. rising, falling or both).
      mask init: same as h16k_ver110_1080/edge_detect
      settings: AttributesFormatString=|
      | rising edges
      | active high
      mask Help: Output is active for one-cycle after each edge of the specified type (i.e. rising, falling, or both).  Latency is zero.
      mask TypeOptions edge: Rising | Falling | Both
      mask TypeOptions polarity: Active High | Active Low
      mask Display:
      | plot(x_in_num,0.5+y_in_num*0.2);
      | plot(x_out_num,0.5+y_out_num*0.2);
  edge_detect2 : Subsystem  AncestorBlock=casper_library_misc/edge_detect  mask(edge_detect){edge=Rising, polarity=Active High, x_in=[0 0.08 0.08 0.16 0.16 0.24 0.24 0.32 0.32 0.4], y_in=[-1 -1  1  1  1  1  1  1  1  1], x_out=[0.6 0.68 0.68 0.76 0.76 0.84 0.84 0.92 0.92 1], y_out=[-1 -1  1  1 -1 -1 -1 -1 -1 -1]}
      mask prompts: edge "Edge Type"; polarity "Output Polarity"; x_in "Input X Positions"; y_in "Input Y Positions"; x_out "Output X Positions"; y_out "Output Y Positions"
      mask help: Output is active for one-cycle after each edge of the specified type (i.e. rising, falling or both).
      mask init: same as h16k_ver110_1080/edge_detect
      settings: AttributesFormatString=|
      | rising edges
      | active high
      mask Help: Output is active for one-cycle after each edge of the specified type (i.e. rising, falling, or both).  Latency is zero.
      mask TypeOptions edge: Rising | Falling | Both
      mask TypeOptions polarity: Active High | Active Low
      mask Display:
      | plot(x_in_num,0.5+y_in_num*0.2);
      | plot(x_out_num,0.5+y_out_num*0.2);
  edge_detect3 : Subsystem  AncestorBlock=casper_library_misc/edge_detect  mask(edge_detect){edge=Falling, polarity=Active High, x_in=[0 0.08 0.08 0.16 0.16 0.24 0.24 0.32 0.32 0.4], y_in=[1  1 -1 -1 -1 -1 -1 -1 -1 -1], x_out=[0.6 0.68 0.68 0.76 0.76 0.84 0.84 0.92 0.92 1], y_out=[-1 -1  1  1 -1 -1 -1 -1 -1 -1]}
      mask prompts: edge "Edge Type"; polarity "Output Polarity"; x_in "Input X Positions"; y_in "Input Y Positions"; x_out "Output X Positions"; y_out "Output Y Positions"
      mask help: Output is active for one-cycle after each edge of the specified type (i.e. rising, falling or both).
      mask init: same as h16k_ver110_1080/edge_detect
      settings: AttributesFormatString=|
      | falling edges
      | active high
      mask Help: Output is active for one-cycle after each edge of the specified type (i.e. rising, falling, or both).  Latency is zero.
      mask TypeOptions edge: Rising | Falling | Both
      mask TypeOptions polarity: Active High | Active Low
      mask Display:
      | plot(x_in_num,0.5+y_in_num*0.2);
      | plot(x_out_num,0.5+y_out_num*0.2);
  edge_detect4 : Subsystem  AncestorBlock=casper_library_misc/edge_detect  mask(edge_detect){edge=Falling, polarity=Active High, x_in=[0 0.08 0.08 0.16 0.16 0.24 0.24 0.32 0.32 0.4], y_in=[1  1 -1 -1 -1 -1 -1 -1 -1 -1], x_out=[0.6 0.68 0.68 0.76 0.76 0.84 0.84 0.92 0.92 1], y_out=[-1 -1  1  1 -1 -1 -1 -1 -1 -1]}
      mask prompts: edge "Edge Type"; polarity "Output Polarity"; x_in "Input X Positions"; y_in "Input Y Positions"; x_out "Output X Positions"; y_out "Output Y Positions"
      mask help: Output is active for one-cycle after each edge of the specified type (i.e. rising, falling or both).
      mask init: same as h16k_ver110_1080/edge_detect
      settings: AttributesFormatString=|
      | falling edges
      | active high
      mask Help: Output is active for one-cycle after each edge of the specified type (i.e. rising, falling, or both).  Latency is zero.
      mask TypeOptions edge: Rising | Falling | Both
      mask TypeOptions polarity: Active High | Active Low
      mask Display:
      | plot(x_in_num,0.5+y_in_num*0.2);
      | plot(x_out_num,0.5+y_out_num*0.2);
  edge_detect5 : Subsystem  AncestorBlock=casper_library_misc/edge_detect  mask(edge_detect){edge=Rising, polarity=Active High, x_in=[0 0.08 0.08 0.16 0.16 0.24 0.24 0.32 0.32 0.4], y_in=[-1 -1  1  1  1  1  1  1  1  1], x_out=[0.6 0.68 0.68 0.76 0.76 0.84 0.84 0.92 0.92 1], y_out=[-1 -1  1  1 -1 -1 -1 -1 -1 -1]}
      mask prompts: edge "Edge Type"; polarity "Output Polarity"; x_in "Input X Positions"; y_in "Input Y Positions"; x_out "Output X Positions"; y_out "Output Y Positions"
      mask help: Output is active for one-cycle after each edge of the specified type (i.e. rising, falling or both).
      mask init: same as h16k_ver110_1080/edge_detect
      settings: AttributesFormatString=|
      | rising edges
      | active high
      mask Help: Output is active for one-cycle after each edge of the specified type (i.e. rising, falling, or both).  Latency is zero.
      mask TypeOptions edge: Rising | Falling | Both
      mask TypeOptions polarity: Active High | Active Low
      mask Display:
      | plot(x_in_num,0.5+y_in_num*0.2);
      | plot(x_out_num,0.5+y_out_num*0.2);
  edge_detect6 : Subsystem  AncestorBlock=casper_library_misc/edge_detect  mask(edge_detect){edge=Rising, polarity=Active High, x_in=[0 0.08 0.08 0.16 0.16 0.24 0.24 0.32 0.32 0.4], y_in=[-1 -1  1  1  1  1  1  1  1  1], x_out=[0.6 0.68 0.68 0.76 0.76 0.84 0.84 0.92 0.92 1], y_out=[-1 -1  1  1 -1 -1 -1 -1 -1 -1]}
      mask prompts: edge "Edge Type"; polarity "Output Polarity"; x_in "Input X Positions"; y_in "Input Y Positions"; x_out "Output X Positions"; y_out "Output Y Positions"
      mask help: Output is active for one-cycle after each edge of the specified type (i.e. rising, falling or both).
      mask init: same as h16k_ver110_1080/edge_detect
      settings: AttributesFormatString=|
      | rising edges
      | active high
      mask Help: Output is active for one-cycle after each edge of the specified type (i.e. rising, falling, or both).  Latency is zero.
      mask TypeOptions edge: Rising | Falling | Both
      mask TypeOptions polarity: Active High | Active Low
      mask Display:
      | plot(x_in_num,0.5+y_in_num*0.2);
      | plot(x_out_num,0.5+y_out_num*0.2);
  err_clear_sim1 : Constant  Value=0
  err_clear_sim3 : Constant  Value=0
  fft_pcore : xps_library/pcore  Tag=xps:pcore  pcore_path=./fftwbr_core/fftwbr_core_ver101.ngc
  fftshift : Subsystem  Tag=xps:sw_reg  AncestorBlock=xps_library/software register  mask(swreg){mode=one value, io_dir=From Processor, io_delay=0, sample_period=1, names=reg, bitwidths=32, arith_types=0, bin_pts=0, sim_port=on, show_format=off}
      mask prompts: io_dir "I/O direction"; io_delay "I/O delay"; sample_period "Sample period"; names "Name:"; bitwidths "Bitwidth:"; arith_types "Type (ufix=0, fix=1, bool=2):"; bin_pts "Binary pt:"; sim_port "Provide sim input/output?"; show_format "Print format string?"
      mask init:
      | swreg_init(gcb)
      settings: AttributesFormatString=1input
      mask TypeOptions mode: one value | fields of equal size | fields of arbitrary size
      mask Callback mode: swreg_cb(gcb);
      mask TypeOptions io_dir: To Processor | From Processor
      mask Callback io_dir:
      | mask_enables = get_param(gcb, 'MaskEnables');
      | mask_names = get_param(gcb, 'MaskNames');
      | if strcmp(get_param(gcb, 'io_dir'), 'To Processor'),
      |     mask_enables{ismember(mask_names, 'sample_period')} = 'off';
      | else
      |     mask_enables{ismember(mask_names, 'sample_period')} = 'on';
      | end
      | set_param(gcb, 'MaskEnables', mask_enables);
      mask Callback bitwidths:
      | swreg_maskcheck(gcb);
      | % blk = gcb;
      | % mode = get_param(blk, 'mode');
      | % current_widths = eval(get_param(blk, 'bitwidths'));
      | % if (strcmp(mode, 'one value') || strcmp(mode, 'fields of equal size')) && (length(current_widths) > 1),
      | %     error('Only one width may be specified for this mode.');
      | % elseif strcmp(mode, 'fields of arbitrary size')
      | %     current_names = textscan(strtrim(strrep(strrep(get_param(blk, 'names'), ']', ''), '[', '')), '%s');
      | %     current_names = current_names{1};
      | %     numios = length(current_names);
      | %     if length(current_widths) ~= numios,
      | %         error('%d field names specified, but %d widths?', numios, length(current_widths));
      | %     end
      | % end
      | % total_width = 0;
      | % for ctr = 1 : length(current_widths),
      | %     total_width = total_width + current_widths(ctr);
      | % end
      | % if total_width > 32,
      | %     error('Total width must be 32 or less, set to %d.', total_width);
      | % end
      mask Callback arith_types:
      | [numios, ~, ~, ~, current_types] = swreg_maskcheck(gcb);
      | % blk = gcb;
      | % mode = get_param(blk, 'mode');
      | % current_types = eval(get_param(blk, 'arith_types'));
      | % numios = length(current_types);
      | % if (strcmp(mode, 'one value') || strcmp(mode, 'fields of equal size')) && (length(current_types) > 1),
      | %     error('Only one type may be specified for this mode.');
      | % elseif strcmp(mode, 'fields of arbitrary size')
      | %     current_names = textscan(strtrim(strrep(strrep(get_param(blk, 'names'), ']', ''), '[', '')), '%s');
      | %     current_names = current_names{1};
      | %     numios = length(current_names);
      | %     if length(current_types) ~= numios,
      | %         error('%d field names specified, but %d types?', numios, length(current_types));
      | %     end
      | % end
      | problem = 0;
      | for ctr = 1 : numios,
      |     t = current_types(ctr);
      |     if (t < 0) || (t > 2),
      |         problem = t;
      |         ctr = numios + 1;
      |     end
      | end
      | if problem ~= 0,
      |     error('Type cannot be %i, must be 0, 1 or 2.', problem);
      | end
      mask Callback bin_pts:
      | swreg_maskcheck(gcb);
      | % blk = gcb;
      | % mode = get_param(blk, 'mode');
      | % current_bins = eval(get_param(blk, 'bin_pts'));
      | % if (strcmp(mode, 'one value') || strcmp(mode, 'fields of equal size')) && (length(current_bins) > 1),
      | %     error('Only one binary pt may be specified for this mode.');
      | % elseif strcmp(mode, 'fields of arbitrary size')
      | %     current_names = textscan(strtrim(strrep(strrep(get_param(blk, 'names'), ']', ''), '[', '')), '%s');
      | %     current_names = current_names{1};
      | %     numios = length(current_names);
      | %     if length(current_bins) ~= numios,
      | %         error('%d field names specified, but %d binary pts?', numios, length(current_bins));
      | %     end
      | % end
  fftwbr_15stages : xbsIndex_r4/Black Box  init_code=fftwbr_core_ver101_config  sim_method=Inactive  verbose=off  block_type=blackbox2
  fftwbr_15stages1 : xbsIndex_r4/Black Box  init_code=fftwbr_core_ver101_config  sim_method=Inactive  verbose=off  block_type=blackbox2
  gbe0 : xps_library/ten_Gbe_v2  Tag=xps:tengbe_v2  flavour=sfp+  slot=1  port_r1=0  port_r2_cx4=0  port_r2_sfpp=0  rx_dist_ram=on  large_frames=on  show_param=on  pre_emph_r2=0.74  pre_emph=3  post_emph_r2=0.18  rxeqmix_r2=7  swing_r2=940  swing=800  fab_en=off  fab_mac=hex2dec('123456780000')  fab_ip=10*(2^24) + 0*(2^16) + 0*(2^8) + 140*(2^0)  fab_udp=60001  fab_gate=1  cpu_rx_en=on  cpu_tx_en=on  ttl=hex2dec('FF')  txctr=off  txerrctr=off  txerrctr_len=100  txofctr=off  txfullctr=off  txvldctr=off  txsnaplen=0 - no snap  rxctr=off  rxerrctr=off  rxerrctr_len=100  rxofctr=off  rxbadctr=off  rxvldctr=off  rxeofctr=off  rxsnaplen=0 - no snap
  manrst : Subsystem  Tag=xps:sw_reg  AncestorBlock=xps_library/software register  mask(swreg){mode=one value, io_dir=From Processor, io_delay=0, sample_period=1, names=reg, bitwidths=32, arith_types=0, bin_pts=0, sim_port=on, show_format=off}
      mask prompts: io_dir "I/O direction"; io_delay "I/O delay"; sample_period "Sample period"; names "Name:"; bitwidths "Bitwidth:"; arith_types "Type (ufix=0, fix=1, bool=2):"; bin_pts "Binary pt:"; sim_port "Provide sim input/output?"; show_format "Print format string?"
      mask init:
      | swreg_init(gcb)
      settings: AttributesFormatString=1input
      mask TypeOptions mode: one value | fields of equal size | fields of arbitrary size
      mask Callback mode: swreg_cb(gcb);
      mask TypeOptions io_dir: To Processor | From Processor
      mask Callback io_dir:
      | mask_enables = get_param(gcb, 'MaskEnables');
      | mask_names = get_param(gcb, 'MaskNames');
      | if strcmp(get_param(gcb, 'io_dir'), 'To Processor'),
      |     mask_enables{ismember(mask_names, 'sample_period')} = 'off';
      | else
      |     mask_enables{ismember(mask_names, 'sample_period')} = 'on';
      | end
      | set_param(gcb, 'MaskEnables', mask_enables);
      mask Callback bitwidths:
      | swreg_maskcheck(gcb);
      | % blk = gcb;
      | % mode = get_param(blk, 'mode');
      | % current_widths = eval(get_param(blk, 'bitwidths'));
      | % if (strcmp(mode, 'one value') || strcmp(mode, 'fields of equal size')) && (length(current_widths) > 1),
      | %     error('Only one width may be specified for this mode.');
      | % elseif strcmp(mode, 'fields of arbitrary size')
      | %     current_names = textscan(strtrim(strrep(strrep(get_param(blk, 'names'), ']', ''), '[', '')), '%s');
      | %     current_names = current_names{1};
      | %     numios = length(current_names);
      | %     if length(current_widths) ~= numios,
      | %         error('%d field names specified, but %d widths?', numios, length(current_widths));
      | %     end
      | % end
      | % total_width = 0;
      | % for ctr = 1 : length(current_widths),
      | %     total_width = total_width + current_widths(ctr);
      | % end
      | % if total_width > 32,
      | %     error('Total width must be 32 or less, set to %d.', total_width);
      | % end
      mask Callback arith_types:
      | [numios, ~, ~, ~, current_types] = swreg_maskcheck(gcb);
      | % blk = gcb;
      | % mode = get_param(blk, 'mode');
      | % current_types = eval(get_param(blk, 'arith_types'));
      | % numios = length(current_types);
      | % if (strcmp(mode, 'one value') || strcmp(mode, 'fields of equal size')) && (length(current_types) > 1),
      | %     error('Only one type may be specified for this mode.');
      | % elseif strcmp(mode, 'fields of arbitrary size')
      | %     current_names = textscan(strtrim(strrep(strrep(get_param(blk, 'names'), ']', ''), '[', '')), '%s');
      | %     current_names = current_names{1};
      | %     numios = length(current_names);
      | %     if length(current_types) ~= numios,
      | %         error('%d field names specified, but %d types?', numios, length(current_types));
      | %     end
      | % end
      | problem = 0;
      | for ctr = 1 : numios,
      |     t = current_types(ctr);
      |     if (t < 0) || (t > 2),
      |         problem = t;
      |         ctr = numios + 1;
      |     end
      | end
      | if problem ~= 0,
      |     error('Type cannot be %i, must be 0, 1 or 2.', problem);
      | end
      mask Callback bin_pts:
      | swreg_maskcheck(gcb);
      | % blk = gcb;
      | % mode = get_param(blk, 'mode');
      | % current_bins = eval(get_param(blk, 'bin_pts'));
      | % if (strcmp(mode, 'one value') || strcmp(mode, 'fields of equal size')) && (length(current_bins) > 1),
      | %     error('Only one binary pt may be specified for this mode.');
      | % elseif strcmp(mode, 'fields of arbitrary size')
      | %     current_names = textscan(strtrim(strrep(strrep(get_param(blk, 'names'), ']', ''), '[', '')), '%s');
      | %     current_names = current_names{1};
      | %     numios = length(current_names);
      | %     if length(current_bins) ~= numios,
      | %         error('%d field names specified, but %d binary pts?', numios, length(current_bins));
      | %     end
      | % end
  npkt : Subsystem  Tag=xps:sw_reg  AncestorBlock=xps_library/software register  mask(swreg){mode=one value, io_dir=To Processor, io_delay=0, sample_period=1, names=reg, bitwidths=32, arith_types=0, bin_pts=0, sim_port=on, show_format=off}
      mask prompts: io_dir "I/O direction"; io_delay "I/O delay"; sample_period "Sample period"; names "Name:"; bitwidths "Bitwidth:"; arith_types "Type (ufix=0, fix=1, bool=2):"; bin_pts "Binary pt:"; sim_port "Provide sim input/output?"; show_format "Print format string?"
      mask init:
      | swreg_init(gcb)
      settings: AttributesFormatString=1output
      mask TypeOptions mode: one value | fields of equal size | fields of arbitrary size
      mask Callback mode: swreg_cb(gcb);
      mask TypeOptions io_dir: To Processor | From Processor
      mask Callback io_dir:
      | mask_enables = get_param(gcb, 'MaskEnables');
      | mask_names = get_param(gcb, 'MaskNames');
      | if strcmp(get_param(gcb, 'io_dir'), 'To Processor'),
      |     mask_enables{ismember(mask_names, 'sample_period')} = 'off';
      | else
      |     mask_enables{ismember(mask_names, 'sample_period')} = 'on';
      | end
      | set_param(gcb, 'MaskEnables', mask_enables);
      mask Callback bitwidths:
      | swreg_maskcheck(gcb);
      | % blk = gcb;
      | % mode = get_param(blk, 'mode');
      | % current_widths = eval(get_param(blk, 'bitwidths'));
      | % if (strcmp(mode, 'one value') || strcmp(mode, 'fields of equal size')) && (length(current_widths) > 1),
      | %     error('Only one width may be specified for this mode.');
      | % elseif strcmp(mode, 'fields of arbitrary size')
      | %     current_names = textscan(strtrim(strrep(strrep(get_param(blk, 'names'), ']', ''), '[', '')), '%s');
      | %     current_names = current_names{1};
      | %     numios = length(current_names);
      | %     if length(current_widths) ~= numios,
      | %         error('%d field names specified, but %d widths?', numios, length(current_widths));
      | %     end
      | % end
      | % total_width = 0;
      | % for ctr = 1 : length(current_widths),
      | %     total_width = total_width + current_widths(ctr);
      | % end
      | % if total_width > 32,
      | %     error('Total width must be 32 or less, set to %d.', total_width);
      | % end
      mask Callback arith_types:
      | [numios, ~, ~, ~, current_types] = swreg_maskcheck(gcb);
      | % blk = gcb;
      | % mode = get_param(blk, 'mode');
      | % current_types = eval(get_param(blk, 'arith_types'));
      | % numios = length(current_types);
      | % if (strcmp(mode, 'one value') || strcmp(mode, 'fields of equal size')) && (length(current_types) > 1),
      | %     error('Only one type may be specified for this mode.');
      | % elseif strcmp(mode, 'fields of arbitrary size')
      | %     current_names = textscan(strtrim(strrep(strrep(get_param(blk, 'names'), ']', ''), '[', '')), '%s');
      | %     current_names = current_names{1};
      | %     numios = length(current_names);
      | %     if length(current_types) ~= numios,
      | %         error('%d field names specified, but %d types?', numios, length(current_types));
      | %     end
      | % end
      | problem = 0;
      | for ctr = 1 : numios,
      |     t = current_types(ctr);
      |     if (t < 0) || (t > 2),
      |         problem = t;
      |         ctr = numios + 1;
      |     end
      | end
      | if problem ~= 0,
      |     error('Type cannot be %i, must be 0, 1 or 2.', problem);
      | end
      mask Callback bin_pts:
      | swreg_maskcheck(gcb);
      | % blk = gcb;
      | % mode = get_param(blk, 'mode');
      | % current_bins = eval(get_param(blk, 'bin_pts'));
      | % if (strcmp(mode, 'one value') || strcmp(mode, 'fields of equal size')) && (length(current_bins) > 1),
      | %     error('Only one binary pt may be specified for this mode.');
      | % elseif strcmp(mode, 'fields of arbitrary size')
      | %     current_names = textscan(strtrim(strrep(strrep(get_param(blk, 'names'), ']', ''), '[', '')), '%s');
      | %     current_names = current_names{1};
      | %     numios = length(current_names);
      | %     if length(current_bins) ~= numios,
      | %         error('%d field names specified, but %d binary pts?', numios, length(current_bins));
      | %     end
      | % end
  nspec : Subsystem  Tag=xps:sw_reg  AncestorBlock=xps_library/software register  mask(swreg){mode=one value, io_dir=To Processor, io_delay=0, sample_period=1, names=reg, bitwidths=32, arith_types=0, bin_pts=0, sim_port=on, show_format=off}
      mask prompts: io_dir "I/O direction"; io_delay "I/O delay"; sample_period "Sample period"; names "Name:"; bitwidths "Bitwidth:"; arith_types "Type (ufix=0, fix=1, bool=2):"; bin_pts "Binary pt:"; sim_port "Provide sim input/output?"; show_format "Print format string?"
      mask init:
      | swreg_init(gcb)
      settings: AttributesFormatString=1output
      mask TypeOptions mode: one value | fields of equal size | fields of arbitrary size
      mask Callback mode: swreg_cb(gcb);
      mask TypeOptions io_dir: To Processor | From Processor
      mask Callback io_dir:
      | mask_enables = get_param(gcb, 'MaskEnables');
      | mask_names = get_param(gcb, 'MaskNames');
      | if strcmp(get_param(gcb, 'io_dir'), 'To Processor'),
      |     mask_enables{ismember(mask_names, 'sample_period')} = 'off';
      | else
      |     mask_enables{ismember(mask_names, 'sample_period')} = 'on';
      | end
      | set_param(gcb, 'MaskEnables', mask_enables);
      mask Callback bitwidths:
      | swreg_maskcheck(gcb);
      | % blk = gcb;
      | % mode = get_param(blk, 'mode');
      | % current_widths = eval(get_param(blk, 'bitwidths'));
      | % if (strcmp(mode, 'one value') || strcmp(mode, 'fields of equal size')) && (length(current_widths) > 1),
      | %     error('Only one width may be specified for this mode.');
      | % elseif strcmp(mode, 'fields of arbitrary size')
      | %     current_names = textscan(strtrim(strrep(strrep(get_param(blk, 'names'), ']', ''), '[', '')), '%s');
      | %     current_names = current_names{1};
      | %     numios = length(current_names);
      | %     if length(current_widths) ~= numios,
      | %         error('%d field names specified, but %d widths?', numios, length(current_widths));
      | %     end
      | % end
      | % total_width = 0;
      | % for ctr = 1 : length(current_widths),
      | %     total_width = total_width + current_widths(ctr);
      | % end
      | % if total_width > 32,
      | %     error('Total width must be 32 or less, set to %d.', total_width);
      | % end
      mask Callback arith_types:
      | [numios, ~, ~, ~, current_types] = swreg_maskcheck(gcb);
      | % blk = gcb;
      | % mode = get_param(blk, 'mode');
      | % current_types = eval(get_param(blk, 'arith_types'));
      | % numios = length(current_types);
      | % if (strcmp(mode, 'one value') || strcmp(mode, 'fields of equal size')) && (length(current_types) > 1),
      | %     error('Only one type may be specified for this mode.');
      | % elseif strcmp(mode, 'fields of arbitrary size')
      | %     current_names = textscan(strtrim(strrep(strrep(get_param(blk, 'names'), ']', ''), '[', '')), '%s');
      | %     current_names = current_names{1};
      | %     numios = length(current_names);
      | %     if length(current_types) ~= numios,
      | %         error('%d field names specified, but %d types?', numios, length(current_types));
      | %     end
      | % end
      | problem = 0;
      | for ctr = 1 : numios,
      |     t = current_types(ctr);
      |     if (t < 0) || (t > 2),
      |         problem = t;
      |         ctr = numios + 1;
      |     end
      | end
      | if problem ~= 0,
      |     error('Type cannot be %i, must be 0, 1 or 2.', problem);
      | end
      mask Callback bin_pts:
      | swreg_maskcheck(gcb);
      | % blk = gcb;
      | % mode = get_param(blk, 'mode');
      | % current_bins = eval(get_param(blk, 'bin_pts'));
      | % if (strcmp(mode, 'one value') || strcmp(mode, 'fields of equal size')) && (length(current_bins) > 1),
      | %     error('Only one binary pt may be specified for this mode.');
      | % elseif strcmp(mode, 'fields of arbitrary size')
      | %     current_names = textscan(strtrim(strrep(strrep(get_param(blk, 'names'), ']', ''), '[', '')), '%s');
      | %     current_names = current_names{1};
      | %     numios = length(current_names);
      | %     if length(current_bins) ~= numios,
      | %         error('%d field names specified, but %d binary pts?', numios, length(current_bins));
      | %     end
      | % end
  pfb_pcore : xps_library/pcore  Tag=xps:pcore  pcore_path=./pfbfirr_core/pfbfirr_core.ngc
  pfbfirr_15stages : xbsIndex_r4/Black Box  init_code=pfbfirr_core_config  sim_method=Inactive  verbose=off  block_type=blackbox2
  pfbfirr_15stages1 : xbsIndex_r4/Black Box  init_code=pfbfirr_core_config  sim_method=Inactive  verbose=off  block_type=blackbox2
  pkt_cntr1 : xbsIndex_r4/Counter  cnt_type=Free Running  cnt_to=Inf  operation=Up  start_count=0  cnt_by_val=1  arith_type=Unsigned  n_bits=32  bin_pt=0  load_pin=off  rst=on  en=on  explicit_period=on  period=1  dbl_ovrd=off  use_behavioral_HDL=off  implementation=Fabric  block_type=counter
      settings: block_version=11.4
  reinterp_vacc{,1..31} (32 alike) : xbsIndex_r4/Reinterpret  force_arith_type=on  arith_type="Signed  (2's comp)"  force_bin_pt=off  bin_pt=0  block_type=reinterpret
  reshaper : Subsystem  mask{inwid=1024, inlen=2048, outwid=64, outchunk=1024, headlen=2000}
      mask prompts: inwid "Input Width (bits)"; inlen "Input Length (clocks)"; outwid "Output Width (bits)"; outchunk "Output Chunk Length (clocks)"; headlen "Header Length"
      mask help:
      | This block takes wide input data and reshapes it to a narrower (or the same)
      | bit width, and breaks it into packets, between which a header can be inserted.
      | Each input data frame must be proceeded by a reset pulse. The input data can be
      | disjoint, with a pulsed valid signal. When the reset signal is pulsed, the previous data
      | frame will be read out. Therefore the number of clocks to read out the header and
      | data must be greater than the number of clocks between two frames (rst signals).
      |
      | The sel signal can be used to drive the select input of a mux which muxes between
      | the data stream (dout) and the indicated number of header words. The header_valid_out
      | signal goes high for each word of the header. dout should be connected to input
      | 0 of the mux. The data_valid_out goes high for each output data value. The st output
      | is for debug access to the internal state machine state.
      mask init:
      | l2inlen = ceil(log2(inlen))
      | l2outchunk = ceil(log2(outchunk))
      | outlen = inlen*(inwid/outwid)
      | nchunk = outlen/outchunk
      | l2headlen = ceil(log2(headlen))
      | l2outlen = ceil(log2(outlen))
  rshpout : Subsystem  Tag=casper:snapshot  AncestorBlock=casper_library_scopes/snapshot  mask(snapshot){storage=bram, dram_dimm=1, dram_clock=200, nsamples=16, data_width=32, offset=off, circap=off, value=off, use_dsp48=on}
      mask prompts: storage "Storage medium"; dram_dimm "DRAM dimm"; dram_clock "DRAM clock rate"; nsamples "Number of Samples (2^?)"; data_width "Data width"; offset "Start delay support"; circap "Circular capture support"; value "Extra value capture support"; use_dsp48 "Use DSP48s to implement counters"
      mask help:
      | Standard snap block, but with the following optional extras;
      |  1) Optionally delay the fabric trigger by a user-specified number of valids.
      |  2) Capture continuously after a trigger until a stop pulse is received. Data is captured into BRAM continuously, with old data being overwritten until a stop command is received. Then stop capturing when memory is filled. This enables you to get some data before and some data after the stop pulse. Use the 'tr_en_cnt' register to determine where you are in your vector. 'Addr' register's MSb now indicates 'busy capturing'.
      |  3) Optionally capture a value on an input port to a register at the same time as the first data sample.
      |  4) Implement counters using DSP48Es to save resources.
      mask init: same as h16k_ver110_1080/adcsnap0
      mask TypeOptions storage: bram | dram
      mask Callback storage: snapshot_callback();
      mask TypeOptions dram_dimm: 1 | 2 | 3 | 4
      mask TypeOptions dram_clock: 200 | 250 | 266 | 300 | 333
      mask TypeOptions data_width: 8 | 16 | 32 | 64 | 128
  sg : Subsystem
  speader1 : Subsystem  mask{spead_msw=64, spead_lsw=40, num_items=6, num_payloads=32}
      mask prompts: num_items "Number of items (+5)"; num_payloads "number of payloads"
      mask help:
      | The size of the heap and payload are in Bytes.
      | If there is one packet per heap then payload_offset is 0.
      | All the input must be not longer than 40 bits.
  spectrum_cntr : xbsIndex_r4/Counter  cnt_type=Free Running  cnt_to=Inf  operation=Up  start_count=0  cnt_by_val=1  arith_type=Unsigned  n_bits=40  bin_pt=0  load_pin=off  rst=on  en=on  explicit_period=on  period=1  dbl_ovrd=off  use_behavioral_HDL=off  implementation=Fabric  block_type=counter
      settings: block_version=11.4
  ssg : Subsystem
  status : Subsystem  Tag=xps:sw_reg  AncestorBlock=xps_library/software register  mask(swreg){mode=one value, io_dir=To Processor, io_delay=0, sample_period=1, names=reg, bitwidths=16, arith_types=0, bin_pts=0, sim_port=on, show_format=off}
      mask prompts: io_dir "I/O direction"; io_delay "I/O delay"; sample_period "Sample period"; names "Name:"; bitwidths "Bitwidth:"; arith_types "Type (ufix=0, fix=1, bool=2):"; bin_pts "Binary pt:"; sim_port "Provide sim input/output?"; show_format "Print format string?"
      mask init:
      | swreg_init(gcb)
      settings: AttributesFormatString=1output
      mask TypeOptions mode: one value | fields of equal size | fields of arbitrary size
      mask Callback mode: swreg_cb(gcb);
      mask TypeOptions io_dir: To Processor | From Processor
      mask Callback io_dir:
      | mask_enables = get_param(gcb, 'MaskEnables');
      | mask_names = get_param(gcb, 'MaskNames');
      | if strcmp(get_param(gcb, 'io_dir'), 'To Processor'),
      |     mask_enables{ismember(mask_names, 'sample_period')} = 'off';
      | else
      |     mask_enables{ismember(mask_names, 'sample_period')} = 'on';
      | end
      | set_param(gcb, 'MaskEnables', mask_enables);
      mask Callback bitwidths:
      | swreg_maskcheck(gcb);
      | % blk = gcb;
      | % mode = get_param(blk, 'mode');
      | % current_widths = eval(get_param(blk, 'bitwidths'));
      | % if (strcmp(mode, 'one value') || strcmp(mode, 'fields of equal size')) && (length(current_widths) > 1),
      | %     error('Only one width may be specified for this mode.');
      | % elseif strcmp(mode, 'fields of arbitrary size')
      | %     current_names = textscan(strtrim(strrep(strrep(get_param(blk, 'names'), ']', ''), '[', '')), '%s');
      | %     current_names = current_names{1};
      | %     numios = length(current_names);
      | %     if length(current_widths) ~= numios,
      | %         error('%d field names specified, but %d widths?', numios, length(current_widths));
      | %     end
      | % end
      | % total_width = 0;
      | % for ctr = 1 : length(current_widths),
      | %     total_width = total_width + current_widths(ctr);
      | % end
      | % if total_width > 32,
      | %     error('Total width must be 32 or less, set to %d.', total_width);
      | % end
      mask Callback arith_types:
      | [numios, ~, ~, ~, current_types] = swreg_maskcheck(gcb);
      | % blk = gcb;
      | % mode = get_param(blk, 'mode');
      | % current_types = eval(get_param(blk, 'arith_types'));
      | % numios = length(current_types);
      | % if (strcmp(mode, 'one value') || strcmp(mode, 'fields of equal size')) && (length(current_types) > 1),
      | %     error('Only one type may be specified for this mode.');
      | % elseif strcmp(mode, 'fields of arbitrary size')
      | %     current_names = textscan(strtrim(strrep(strrep(get_param(blk, 'names'), ']', ''), '[', '')), '%s');
      | %     current_names = current_names{1};
      | %     numios = length(current_names);
      | %     if length(current_types) ~= numios,
      | %         error('%d field names specified, but %d types?', numios, length(current_types));
      | %     end
      | % end
      | problem = 0;
      | for ctr = 1 : numios,
      |     t = current_types(ctr);
      |     if (t < 0) || (t > 2),
      |         problem = t;
      |         ctr = numios + 1;
      |     end
      | end
      | if problem ~= 0,
      |     error('Type cannot be %i, must be 0, 1 or 2.', problem);
      | end
      mask Callback bin_pts:
      | swreg_maskcheck(gcb);
      | % blk = gcb;
      | % mode = get_param(blk, 'mode');
      | % current_bins = eval(get_param(blk, 'bin_pts'));
      | % if (strcmp(mode, 'one value') || strcmp(mode, 'fields of equal size')) && (length(current_bins) > 1),
      | %     error('Only one binary pt may be specified for this mode.');
      | % elseif strcmp(mode, 'fields of arbitrary size')
      | %     current_names = textscan(strtrim(strrep(strrep(get_param(blk, 'names'), ']', ''), '[', '')), '%s');
      | %     current_names = current_names{1};
      | %     numios = length(current_names);
      | %     if length(current_bins) ~= numios,
      | %         error('%d field names specified, but %d binary pts?', numios, length(current_bins));
      | %     end
      | % end
  stokesout : Subsystem  Tag=casper:snapshot  AncestorBlock=casper_library_scopes/snapshot  mask(snapshot){storage=bram, dram_dimm=1, dram_clock=200, nsamples=10, data_width=32, offset=off, circap=off, value=off, use_dsp48=on}
      mask prompts: storage "Storage medium"; dram_dimm "DRAM dimm"; dram_clock "DRAM clock rate"; nsamples "Number of Samples (2^?)"; data_width "Data width"; offset "Start delay support"; circap "Circular capture support"; value "Extra value capture support"; use_dsp48 "Use DSP48s to implement counters"
      mask help:
      | Standard snap block, but with the following optional extras;
      |  1) Optionally delay the fabric trigger by a user-specified number of valids.
      |  2) Capture continuously after a trigger until a stop pulse is received. Data is captured into BRAM continuously, with old data being overwritten until a stop command is received. Then stop capturing when memory is filled. This enables you to get some data before and some data after the stop pulse. Use the 'tr_en_cnt' register to determine where you are in your vector. 'Addr' register's MSb now indicates 'busy capturing'.
      |  3) Optionally capture a value on an input port to a register at the same time as the first data sample.
      |  4) Implement counters using DSP48Es to save resources.
      mask init: same as h16k_ver110_1080/adcsnap0
      mask TypeOptions storage: bram | dram
      mask Callback storage: snapshot_callback();
      mask TypeOptions dram_dimm: 1 | 2 | 3 | 4
      mask TypeOptions dram_clock: 200 | 250 | 266 | 300 | 333
      mask TypeOptions data_width: 8 | 16 | 32 | 64 | 128
  time_cntr : xbsIndex_r4/Counter  cnt_type=Free Running  cnt_to=Inf  operation=Up  start_count=0  cnt_by_val=1  arith_type=Unsigned  n_bits=40  bin_pt=0  load_pin=off  rst=on  en=off  explicit_period=on  period=1  dbl_ovrd=off  use_behavioral_HDL=off  implementation=Fabric  block_type=counter
      settings: block_version=11.4
  timesel : Subsystem  Tag=xps:sw_reg  AncestorBlock=xps_library/software register  mask(swreg){mode=one value, io_dir=From Processor, io_delay=0, sample_period=1, names=reg, bitwidths=32, arith_types=0, bin_pts=0, sim_port=on, show_format=off}
      mask prompts: io_dir "I/O direction"; io_delay "I/O delay"; sample_period "Sample period"; names "Name:"; bitwidths "Bitwidth:"; arith_types "Type (ufix=0, fix=1, bool=2):"; bin_pts "Binary pt:"; sim_port "Provide sim input/output?"; show_format "Print format string?"
      mask init:
      | swreg_init(gcb)
      settings: AttributesFormatString=1input
      mask TypeOptions mode: one value | fields of equal size | fields of arbitrary size
      mask Callback mode: swreg_cb(gcb);
      mask TypeOptions io_dir: To Processor | From Processor
      mask Callback io_dir:
      | mask_enables = get_param(gcb, 'MaskEnables');
      | mask_names = get_param(gcb, 'MaskNames');
      | if strcmp(get_param(gcb, 'io_dir'), 'To Processor'),
      |     mask_enables{ismember(mask_names, 'sample_period')} = 'off';
      | else
      |     mask_enables{ismember(mask_names, 'sample_period')} = 'on';
      | end
      | set_param(gcb, 'MaskEnables', mask_enables);
      mask Callback bitwidths:
      | swreg_maskcheck(gcb);
      | % blk = gcb;
      | % mode = get_param(blk, 'mode');
      | % current_widths = eval(get_param(blk, 'bitwidths'));
      | % if (strcmp(mode, 'one value') || strcmp(mode, 'fields of equal size')) && (length(current_widths) > 1),
      | %     error('Only one width may be specified for this mode.');
      | % elseif strcmp(mode, 'fields of arbitrary size')
      | %     current_names = textscan(strtrim(strrep(strrep(get_param(blk, 'names'), ']', ''), '[', '')), '%s');
      | %     current_names = current_names{1};
      | %     numios = length(current_names);
      | %     if length(current_widths) ~= numios,
      | %         error('%d field names specified, but %d widths?', numios, length(current_widths));
      | %     end
      | % end
      | % total_width = 0;
      | % for ctr = 1 : length(current_widths),
      | %     total_width = total_width + current_widths(ctr);
      | % end
      | % if total_width > 32,
      | %     error('Total width must be 32 or less, set to %d.', total_width);
      | % end
      mask Callback arith_types:
      | [numios, ~, ~, ~, current_types] = swreg_maskcheck(gcb);
      | % blk = gcb;
      | % mode = get_param(blk, 'mode');
      | % current_types = eval(get_param(blk, 'arith_types'));
      | % numios = length(current_types);
      | % if (strcmp(mode, 'one value') || strcmp(mode, 'fields of equal size')) && (length(current_types) > 1),
      | %     error('Only one type may be specified for this mode.');
      | % elseif strcmp(mode, 'fields of arbitrary size')
      | %     current_names = textscan(strtrim(strrep(strrep(get_param(blk, 'names'), ']', ''), '[', '')), '%s');
      | %     current_names = current_names{1};
      | %     numios = length(current_names);
      | %     if length(current_types) ~= numios,
      | %         error('%d field names specified, but %d types?', numios, length(current_types));
      | %     end
      | % end
      | problem = 0;
      | for ctr = 1 : numios,
      |     t = current_types(ctr);
      |     if (t < 0) || (t > 2),
      |         problem = t;
      |         ctr = numios + 1;
      |     end
      | end
      | if problem ~= 0,
      |     error('Type cannot be %i, must be 0, 1 or 2.', problem);
      | end
      mask Callback bin_pts:
      | swreg_maskcheck(gcb);
      | % blk = gcb;
      | % mode = get_param(blk, 'mode');
      | % current_bins = eval(get_param(blk, 'bin_pts'));
      | % if (strcmp(mode, 'one value') || strcmp(mode, 'fields of equal size')) && (length(current_bins) > 1),
      | %     error('Only one binary pt may be specified for this mode.');
      | % elseif strcmp(mode, 'fields of arbitrary size')
      | %     current_names = textscan(strtrim(strrep(strrep(get_param(blk, 'names'), ']', ''), '[', '')), '%s');
      | %     current_names = current_names{1};
      | %     numios = length(current_names);
      | %     if length(current_bins) ~= numios,
      | %         error('%d field names specified, but %d binary pts?', numios, length(current_bins));
      | %     end
      | % end
  timesnap : Subsystem  Tag=casper:snapshot  AncestorBlock=casper_library_scopes/snapshot  mask(snapshot){storage=bram, dram_dimm=1, dram_clock=200, nsamples=10, data_width=64, offset=off, circap=off, value=off, use_dsp48=on}
      mask prompts: storage "Storage medium"; dram_dimm "DRAM dimm"; dram_clock "DRAM clock rate"; nsamples "Number of Samples (2^?)"; data_width "Data width"; offset "Start delay support"; circap "Circular capture support"; value "Extra value capture support"; use_dsp48 "Use DSP48s to implement counters"
      mask help:
      | Standard snap block, but with the following optional extras;
      |  1) Optionally delay the fabric trigger by a user-specified number of valids.
      |  2) Capture continuously after a trigger until a stop pulse is received. Data is captured into BRAM continuously, with old data being overwritten until a stop command is received. Then stop capturing when memory is filled. This enables you to get some data before and some data after the stop pulse. Use the 'tr_en_cnt' register to determine where you are in your vector. 'Addr' register's MSb now indicates 'busy capturing'.
      |  3) Optionally capture a value on an input port to a register at the same time as the first data sample.
      |  4) Implement counters using DSP48Es to save resources.
      mask init: same as h16k_ver110_1080/adcsnap0
      mask TypeOptions storage: bram | dram
      mask Callback storage: snapshot_callback();
      mask TypeOptions dram_dimm: 1 | 2 | 3 | 4
      mask TypeOptions dram_clock: 200 | 250 | 266 | 300 | 333
      mask TypeOptions data_width: 8 | 16 | 32 | 64 | 128
  trig : Subsystem  Tag=xps:sw_reg  AncestorBlock=xps_library/software register  mask(swreg){mode=one value, io_dir=From Processor, io_delay=0, sample_period=1, names=reg, bitwidths=32, arith_types=0, bin_pts=0, sim_port=on, show_format=off}
      mask prompts: io_dir "I/O direction"; io_delay "I/O delay"; sample_period "Sample period"; names "Name:"; bitwidths "Bitwidth:"; arith_types "Type (ufix=0, fix=1, bool=2):"; bin_pts "Binary pt:"; sim_port "Provide sim input/output?"; show_format "Print format string?"
      mask init:
      | swreg_init(gcb)
      settings: AttributesFormatString=1input
      mask TypeOptions mode: one value | fields of equal size | fields of arbitrary size
      mask Callback mode: swreg_cb(gcb);
      mask TypeOptions io_dir: To Processor | From Processor
      mask Callback io_dir:
      | mask_enables = get_param(gcb, 'MaskEnables');
      | mask_names = get_param(gcb, 'MaskNames');
      | if strcmp(get_param(gcb, 'io_dir'), 'To Processor'),
      |     mask_enables{ismember(mask_names, 'sample_period')} = 'off';
      | else
      |     mask_enables{ismember(mask_names, 'sample_period')} = 'on';
      | end
      | set_param(gcb, 'MaskEnables', mask_enables);
      mask Callback bitwidths:
      | swreg_maskcheck(gcb);
      | % blk = gcb;
      | % mode = get_param(blk, 'mode');
      | % current_widths = eval(get_param(blk, 'bitwidths'));
      | % if (strcmp(mode, 'one value') || strcmp(mode, 'fields of equal size')) && (length(current_widths) > 1),
      | %     error('Only one width may be specified for this mode.');
      | % elseif strcmp(mode, 'fields of arbitrary size')
      | %     current_names = textscan(strtrim(strrep(strrep(get_param(blk, 'names'), ']', ''), '[', '')), '%s');
      | %     current_names = current_names{1};
      | %     numios = length(current_names);
      | %     if length(current_widths) ~= numios,
      | %         error('%d field names specified, but %d widths?', numios, length(current_widths));
      | %     end
      | % end
      | % total_width = 0;
      | % for ctr = 1 : length(current_widths),
      | %     total_width = total_width + current_widths(ctr);
      | % end
      | % if total_width > 32,
      | %     error('Total width must be 32 or less, set to %d.', total_width);
      | % end
      mask Callback arith_types:
      | [numios, ~, ~, ~, current_types] = swreg_maskcheck(gcb);
      | % blk = gcb;
      | % mode = get_param(blk, 'mode');
      | % current_types = eval(get_param(blk, 'arith_types'));
      | % numios = length(current_types);
      | % if (strcmp(mode, 'one value') || strcmp(mode, 'fields of equal size')) && (length(current_types) > 1),
      | %     error('Only one type may be specified for this mode.');
      | % elseif strcmp(mode, 'fields of arbitrary size')
      | %     current_names = textscan(strtrim(strrep(strrep(get_param(blk, 'names'), ']', ''), '[', '')), '%s');
      | %     current_names = current_names{1};
      | %     numios = length(current_names);
      | %     if length(current_types) ~= numios,
      | %         error('%d field names specified, but %d types?', numios, length(current_types));
      | %     end
      | % end
      | problem = 0;
      | for ctr = 1 : numios,
      |     t = current_types(ctr);
      |     if (t < 0) || (t > 2),
      |         problem = t;
      |         ctr = numios + 1;
      |     end
      | end
      | if problem ~= 0,
      |     error('Type cannot be %i, must be 0, 1 or 2.', problem);
      | end
      mask Callback bin_pts:
      | swreg_maskcheck(gcb);
      | % blk = gcb;
      | % mode = get_param(blk, 'mode');
      | % current_bins = eval(get_param(blk, 'bin_pts'));
      | % if (strcmp(mode, 'one value') || strcmp(mode, 'fields of equal size')) && (length(current_bins) > 1),
      | %     error('Only one binary pt may be specified for this mode.');
      | % elseif strcmp(mode, 'fields of arbitrary size')
      | %     current_names = textscan(strtrim(strrep(strrep(get_param(blk, 'names'), ']', ''), '[', '')), '%s');
      | %     current_names = current_names{1};
      | %     numios = length(current_names);
      | %     if length(current_bins) ~= numios,
      | %         error('%d field names specified, but %d binary pts?', numios, length(current_bins));
      | %     end
      | % end
  vacc0 : Subsystem  AncestorBlock=gavrt_library/vacc  mask(vacc){veclen=11, n_inputs=4, max_accum=10, arith_type=1, in_bit_width=32, in_bin_pt=0, out_bit_width=42, out_bin_pt=0, register_din=1, add_latency=2, bram_latency=2, mux_latency=0, use_dsp48=1}
      mask prompts: veclen "Vector Length (2^?)"; n_inputs "Number of Simultaneous Vectors"; max_accum "Maximum # Accumulations (2^?)"; arith_type "Arithmetic Type (0=Unsigned, 1=Signed)"; in_bit_width "Input Bit Width"; in_bin_pt "Input Binary Point"; out_bit_width "Output Bit Width"; out_bin_pt "Output Binary Point"; register_din "Register Input Data  (1 = Enable Register Retiming on input delay)"; add_latency "Add Latency"; bram_latency "BRAM Latency"; mux_latency "Mux Latency"; use_dsp48 "Use DSP48"
      mask help:
      | Sync is expected the clock before the first data to be accumulated.
      | Use the Cram block to feed din for multiple simultaneous inputs.
      | acc_len is the number of vectors to sum.
      | valid is high while a valid accumulation is being clocked out on dout.
      | If only one sync pulse is provided, valid accumulations will repeatedly appear on dout as they become available.
      | Undesired behavior may occur if acc_len is changed without a new sync pulse.
      | Note: The output is an unsigned concatenation of the output streams. Thus, even with only one stream, the output must be recast before using.
      | Register Input Data controls the "Enable Register Retiming" parameter of the delays on 'din'.
      mask init:
      | config.toplevel = gcb;
      | config.source = str2func('vacc_init_xblock');
      | xBlock( config, {...
      |     'veclen', veclen, ...
      |     'n_inputs', n_inputs, ...
      |     'max_accum', max_accum, ...
      |     'arith_type', arith_type, ...
      |     'in_bit_width', in_bit_width, ...
      |     'in_bin_pt', in_bin_pt, ...
      |     'out_bit_width', out_bit_width, ...
      |     'out_bin_pt', out_bin_pt, ...
      |     'register_din', register_din, ...
      |     'add_latency', add_latency, ...
      |     'bram_latency', bram_latency, ...
      |     'mux_latency', mux_latency, ...
      |     'use_dsp48', use_dsp48, ...
      | });
      settings: AttributesFormatString=|
      | vector length=32, inputs=4
      | max accumulations=2^5
  vacc1 : Subsystem  AncestorBlock=gavrt_library/vacc  mask(vacc){veclen=11, n_inputs=4, max_accum=10, arith_type=1, in_bit_width=32, in_bin_pt=0, out_bit_width=42, out_bin_pt=0, register_din=1, add_latency=2, bram_latency=2, mux_latency=0, use_dsp48=1}
      mask prompts: veclen "Vector Length (2^?)"; n_inputs "Number of Simultaneous Vectors"; max_accum "Maximum # Accumulations (2^?)"; arith_type "Arithmetic Type (0=Unsigned, 1=Signed)"; in_bit_width "Input Bit Width"; in_bin_pt "Input Binary Point"; out_bit_width "Output Bit Width"; out_bin_pt "Output Binary Point"; register_din "Register Input Data  (1 = Enable Register Retiming on input delay)"; add_latency "Add Latency"; bram_latency "BRAM Latency"; mux_latency "Mux Latency"; use_dsp48 "Use DSP48"
      mask help:
      | Sync is expected the clock before the first data to be accumulated.
      | Use the Cram block to feed din for multiple simultaneous inputs.
      | acc_len is the number of vectors to sum.
      | valid is high while a valid accumulation is being clocked out on dout.
      | If only one sync pulse is provided, valid accumulations will repeatedly appear on dout as they become available.
      | Undesired behavior may occur if acc_len is changed without a new sync pulse.
      | Note: The output is an unsigned concatenation of the output streams. Thus, even with only one stream, the output must be recast before using.
      | Register Input Data controls the "Enable Register Retiming" parameter of the delays on 'din'.
      mask init: same as h16k_ver110_1080/vacc0
      settings: AttributesFormatString=|
      | vector length=32, inputs=4
      | max accumulations=2^5
  vacc2 : Subsystem  AncestorBlock=gavrt_library/vacc  mask(vacc){veclen=11, n_inputs=4, max_accum=10, arith_type=1, in_bit_width=32, in_bin_pt=0, out_bit_width=42, out_bin_pt=0, register_din=1, add_latency=2, bram_latency=2, mux_latency=0, use_dsp48=1}
      mask prompts: veclen "Vector Length (2^?)"; n_inputs "Number of Simultaneous Vectors"; max_accum "Maximum # Accumulations (2^?)"; arith_type "Arithmetic Type (0=Unsigned, 1=Signed)"; in_bit_width "Input Bit Width"; in_bin_pt "Input Binary Point"; out_bit_width "Output Bit Width"; out_bin_pt "Output Binary Point"; register_din "Register Input Data  (1 = Enable Register Retiming on input delay)"; add_latency "Add Latency"; bram_latency "BRAM Latency"; mux_latency "Mux Latency"; use_dsp48 "Use DSP48"
      mask help:
      | Sync is expected the clock before the first data to be accumulated.
      | Use the Cram block to feed din for multiple simultaneous inputs.
      | acc_len is the number of vectors to sum.
      | valid is high while a valid accumulation is being clocked out on dout.
      | If only one sync pulse is provided, valid accumulations will repeatedly appear on dout as they become available.
      | Undesired behavior may occur if acc_len is changed without a new sync pulse.
      | Note: The output is an unsigned concatenation of the output streams. Thus, even with only one stream, the output must be recast before using.
      | Register Input Data controls the "Enable Register Retiming" parameter of the delays on 'din'.
      mask init: same as h16k_ver110_1080/vacc0
      settings: AttributesFormatString=|
      | vector length=32, inputs=4
      | max accumulations=2^5
  vacc3 : Subsystem  AncestorBlock=gavrt_library/vacc  mask(vacc){veclen=11, n_inputs=4, max_accum=10, arith_type=1, in_bit_width=32, in_bin_pt=0, out_bit_width=42, out_bin_pt=0, register_din=1, add_latency=2, bram_latency=2, mux_latency=0, use_dsp48=1}
      mask prompts: veclen "Vector Length (2^?)"; n_inputs "Number of Simultaneous Vectors"; max_accum "Maximum # Accumulations (2^?)"; arith_type "Arithmetic Type (0=Unsigned, 1=Signed)"; in_bit_width "Input Bit Width"; in_bin_pt "Input Binary Point"; out_bit_width "Output Bit Width"; out_bin_pt "Output Binary Point"; register_din "Register Input Data  (1 = Enable Register Retiming on input delay)"; add_latency "Add Latency"; bram_latency "BRAM Latency"; mux_latency "Mux Latency"; use_dsp48 "Use DSP48"
      mask help:
      | Sync is expected the clock before the first data to be accumulated.
      | Use the Cram block to feed din for multiple simultaneous inputs.
      | acc_len is the number of vectors to sum.
      | valid is high while a valid accumulation is being clocked out on dout.
      | If only one sync pulse is provided, valid accumulations will repeatedly appear on dout as they become available.
      | Undesired behavior may occur if acc_len is changed without a new sync pulse.
      | Note: The output is an unsigned concatenation of the output streams. Thus, even with only one stream, the output must be recast before using.
      | Register Input Data controls the "Enable Register Retiming" parameter of the delays on 'din'.
      mask init: same as h16k_ver110_1080/vacc0
      settings: AttributesFormatString=|
      | vector length=32, inputs=4
      | max accumulations=2^5
  vacc4 : Subsystem  AncestorBlock=gavrt_library/vacc  mask(vacc){veclen=11, n_inputs=4, max_accum=10, arith_type=1, in_bit_width=32, in_bin_pt=0, out_bit_width=42, out_bin_pt=0, register_din=1, add_latency=2, bram_latency=2, mux_latency=0, use_dsp48=1}
      mask prompts: veclen "Vector Length (2^?)"; n_inputs "Number of Simultaneous Vectors"; max_accum "Maximum # Accumulations (2^?)"; arith_type "Arithmetic Type (0=Unsigned, 1=Signed)"; in_bit_width "Input Bit Width"; in_bin_pt "Input Binary Point"; out_bit_width "Output Bit Width"; out_bin_pt "Output Binary Point"; register_din "Register Input Data  (1 = Enable Register Retiming on input delay)"; add_latency "Add Latency"; bram_latency "BRAM Latency"; mux_latency "Mux Latency"; use_dsp48 "Use DSP48"
      mask help:
      | Sync is expected the clock before the first data to be accumulated.
      | Use the Cram block to feed din for multiple simultaneous inputs.
      | acc_len is the number of vectors to sum.
      | valid is high while a valid accumulation is being clocked out on dout.
      | If only one sync pulse is provided, valid accumulations will repeatedly appear on dout as they become available.
      | Undesired behavior may occur if acc_len is changed without a new sync pulse.
      | Note: The output is an unsigned concatenation of the output streams. Thus, even with only one stream, the output must be recast before using.
      | Register Input Data controls the "Enable Register Retiming" parameter of the delays on 'din'.
      mask init: same as h16k_ver110_1080/vacc0
      settings: AttributesFormatString=|
      | vector length=32, inputs=4
      | max accumulations=2^5
  vacc5 : Subsystem  AncestorBlock=gavrt_library/vacc  mask(vacc){veclen=11, n_inputs=4, max_accum=10, arith_type=1, in_bit_width=32, in_bin_pt=0, out_bit_width=42, out_bin_pt=0, register_din=1, add_latency=2, bram_latency=2, mux_latency=0, use_dsp48=1}
      mask prompts: veclen "Vector Length (2^?)"; n_inputs "Number of Simultaneous Vectors"; max_accum "Maximum # Accumulations (2^?)"; arith_type "Arithmetic Type (0=Unsigned, 1=Signed)"; in_bit_width "Input Bit Width"; in_bin_pt "Input Binary Point"; out_bit_width "Output Bit Width"; out_bin_pt "Output Binary Point"; register_din "Register Input Data  (1 = Enable Register Retiming on input delay)"; add_latency "Add Latency"; bram_latency "BRAM Latency"; mux_latency "Mux Latency"; use_dsp48 "Use DSP48"
      mask help:
      | Sync is expected the clock before the first data to be accumulated.
      | Use the Cram block to feed din for multiple simultaneous inputs.
      | acc_len is the number of vectors to sum.
      | valid is high while a valid accumulation is being clocked out on dout.
      | If only one sync pulse is provided, valid accumulations will repeatedly appear on dout as they become available.
      | Undesired behavior may occur if acc_len is changed without a new sync pulse.
      | Note: The output is an unsigned concatenation of the output streams. Thus, even with only one stream, the output must be recast before using.
      | Register Input Data controls the "Enable Register Retiming" parameter of the delays on 'din'.
      mask init: same as h16k_ver110_1080/vacc0
      settings: AttributesFormatString=|
      | vector length=32, inputs=4
      | max accumulations=2^5
  vacc6 : Subsystem  AncestorBlock=gavrt_library/vacc  mask(vacc){veclen=11, n_inputs=4, max_accum=10, arith_type=1, in_bit_width=32, in_bin_pt=0, out_bit_width=42, out_bin_pt=0, register_din=1, add_latency=2, bram_latency=2, mux_latency=0, use_dsp48=1}
      mask prompts: veclen "Vector Length (2^?)"; n_inputs "Number of Simultaneous Vectors"; max_accum "Maximum # Accumulations (2^?)"; arith_type "Arithmetic Type (0=Unsigned, 1=Signed)"; in_bit_width "Input Bit Width"; in_bin_pt "Input Binary Point"; out_bit_width "Output Bit Width"; out_bin_pt "Output Binary Point"; register_din "Register Input Data  (1 = Enable Register Retiming on input delay)"; add_latency "Add Latency"; bram_latency "BRAM Latency"; mux_latency "Mux Latency"; use_dsp48 "Use DSP48"
      mask help:
      | Sync is expected the clock before the first data to be accumulated.
      | Use the Cram block to feed din for multiple simultaneous inputs.
      | acc_len is the number of vectors to sum.
      | valid is high while a valid accumulation is being clocked out on dout.
      | If only one sync pulse is provided, valid accumulations will repeatedly appear on dout as they become available.
      | Undesired behavior may occur if acc_len is changed without a new sync pulse.
      | Note: The output is an unsigned concatenation of the output streams. Thus, even with only one stream, the output must be recast before using.
      | Register Input Data controls the "Enable Register Retiming" parameter of the delays on 'din'.
      mask init: same as h16k_ver110_1080/vacc0
      settings: AttributesFormatString=|
      | vector length=32, inputs=4
      | max accumulations=2^5
  vacc7 : Subsystem  AncestorBlock=gavrt_library/vacc  mask(vacc){veclen=11, n_inputs=4, max_accum=10, arith_type=1, in_bit_width=32, in_bin_pt=0, out_bit_width=42, out_bin_pt=0, register_din=1, add_latency=2, bram_latency=2, mux_latency=0, use_dsp48=1}
      mask prompts: veclen "Vector Length (2^?)"; n_inputs "Number of Simultaneous Vectors"; max_accum "Maximum # Accumulations (2^?)"; arith_type "Arithmetic Type (0=Unsigned, 1=Signed)"; in_bit_width "Input Bit Width"; in_bin_pt "Input Binary Point"; out_bit_width "Output Bit Width"; out_bin_pt "Output Binary Point"; register_din "Register Input Data  (1 = Enable Register Retiming on input delay)"; add_latency "Add Latency"; bram_latency "BRAM Latency"; mux_latency "Mux Latency"; use_dsp48 "Use DSP48"
      mask help:
      | Sync is expected the clock before the first data to be accumulated.
      | Use the Cram block to feed din for multiple simultaneous inputs.
      | acc_len is the number of vectors to sum.
      | valid is high while a valid accumulation is being clocked out on dout.
      | If only one sync pulse is provided, valid accumulations will repeatedly appear on dout as they become available.
      | Undesired behavior may occur if acc_len is changed without a new sync pulse.
      | Note: The output is an unsigned concatenation of the output streams. Thus, even with only one stream, the output must be recast before using.
      | Register Input Data controls the "Enable Register Retiming" parameter of the delays on 'din'.
      mask init: same as h16k_ver110_1080/vacc0
      settings: AttributesFormatString=|
      | vector length=32, inputs=4
      | max accumulations=2^5
  wires:
  manrst/1(in_reg) -> Register16/1
  Constant19/1 -> manrst/1(sim_1)
  Register16/1 -> Slice2/1, Slice4/1
  Slice2/1 -> Delay26/1
  Register10/1 -> [xout0]
  Register11/1 -> [xout1]
  Register9/1 -> Delay2/1
  Register48/1 -> [yout0]
  Register49/1 -> [yout1]
  Slice10/1 -> edge_detect5/1(in)
  Register44/1 -> Slice10/1
  Constant6/1 -> gbe0/7
  gbe0/10 -> Terminator/1
  gbe0/2 -> Terminator17/1
  gbe0/3 -> Terminator16/1
  gbe0/4 -> Terminator15/1
  gbe0/5 -> [txovf]
  gbe0/6 -> Terminator8/1
  gbe0/7 -> Terminator6/1
  gbe0/8 -> Terminator5/1
  gbe0/9 -> Terminator3/1
  gbe0/11 -> Terminator11/1
  Constant5/1 -> gbe0/8
  Delay21/1 -> gbe0/6
  Delay25/1 -> gbe0/3
  Delay29/1 -> gbe0/2
  Delay30/1 -> gbe0/1
  acc_len/1(in_reg) -> Delay32/1
  Constant3/1 -> acc_len/1(sim_1)
  Delay32/1 -> [acc_len]
  err_clear_sim1/1 -> dest_ip/1(sim_1)
  dest_ip/1(in_reg) -> [dest_ip]
  dest_port/1(in_reg) -> Slice7/1
  err_clear_sim3/1 -> dest_port/1(sim_1)
  Slice7/1 -> [dest_port]
  [tge_rst] -> Delay30/1
  [data_out] -> speader1/1(data_in)
  [data_valid] -> speader1/2(valid_in)
  [dest_ip] -> gbe0/4
  [dest_port] -> gbe0/5
  speader1/3(eof) -> [eof]
  [eof] -> Delay21/1
  Constant18/1 -> speader1/3(heap_size)
  Constant33/1 -> speader1/8(mode)
  Constant34/1 -> speader1/10(payload_offset)
  speader1/2(data_valid) -> [data_valid_spead]
  [data_valid_spead] -> Delay25/1
  [data_spead] -> Delay29/1
  [master_rst1] -> time_cntr/1
  Slice5/1 -> [xxout0]
  Slice6/1 -> [yyout0]
  Slice13/1 -> [xyoutre0]
  Slice18/1 -> [xyoutim0]
  Slice19/1 -> [xxout1]
  Slice20/1 -> [yyout1]
  Slice21/1 -> [xyoutre1]
  Slice22/1 -> [xyoutim1]
  [acc_len] -> Convert/1
  Constant24/1 -> speader1/4(Packet_length)
  [master_rst1] -> spectrum_cntr/1
  [eoh] -> spectrum_cntr/2
  [spead_rst] -> speader1/11(Reset)
  Convert/1 -> speader1/7(integration size)
  speader1/1(data_out) -> [data_spead]
  [fftshift] -> Delay5/1
  Register1/1 -> [xout2]
  Register2/1 -> [xout3]
  Register12/1 -> [yout2]
  Register13/1 -> [yout3]
  Slice29/1 -> [xxout2]
  Slice30/1 -> [yyout2]
  Slice14/1 -> [xyoutre2]
  Slice15/1 -> [xyoutim2]
  Slice25/1 -> [xxout3]
  Slice26/1 -> [yyout3]
  Slice27/1 -> [xyoutre3]
  Slice28/1 -> [xyoutim3]
  spectrum_cntr/1 -> [spec_cntr]
  time_cntr/1 -> [time_cntr]
  [time_cntr] -> speader1/5(time_stamp)
  [spec_cntr] -> speader1/6(spectrum counter)
  cram4/1(Out) -> [din]
  speader1/4(eoh) -> [eoh]
  reshaper/2(sel) -> Terminator10/1
  reshaper/3(header_valid_out) -> Terminator13/1
  [din] -> Delay13/1
  Delay10/1 -> Delay11/1, edge_detect4/1(in)
  Delay13/1 -> Delay12/1
  Delay12/1 -> reshaper/3(din)
  Delay11/1 -> reshaper/2(valid)
  reshaper/5(st) -> [reshape_state]
  Delay14/1 -> Slice41/1, [data_out]
  Delay15/1 -> [data_valid], Counter2/1, edge_detect6/1(in), Delay41/1
  reshaper/1(dout) -> Delay14/1
  reshaper/4(data_valid_out) -> Delay15/1
  Constant30/1 -> Register19/1
  Register18/1 -> Inverter/1
  Inverter/1 -> Register19/2, [spead_rst]  "ppsready"
  Constant31/1 -> Register18/1
  arm/1(in_reg) -> Register20/1
  Constant12/1 -> arm/1(sim_1)
  Register20/1 -> Slice3/1
  Slice3/1 -> [arm]
  [arm] -> Register18/2
  [master_rst2] -> Register18/3
  [sync_out] -> Register19/3
  Register19/1 -> [data_enable]
  [valid] -> Logical/1
  [data_enable] -> Logical/2
  Logical/1 -> Delay10/1
  Delay4/1 -> speader1/9(status_bits)
  [fftshift] -> Delay6/1
  [adc_sync] -> sg/1(pps)
  gbe0/1 -> Terminator9/1, [ledup]
  Slice4/1 -> [auto_reset_enable]
  [arm] -> edge_detect2/1(in)
  edge_detect2/1(out) -> Delay60/1
  Logical2/1 -> [tge_rst]
  Delay26/1 -> Logical2/1
  Logical3/1 -> Logical2/3
  [auto_reset_enable] -> Logical3/1
  [txovf] -> edge_detect1/1(in)
  edge_detect1/1(out) -> Logical3/2
  [master_rst4] -> Counter1/1
  Counter1/1 -> Slice8/1
  Slice8/1 -> edge_detect3/1(in)
  edge_detect3/1(out) -> [spec_tick]
  Constant10/1 -> bus_create2/1(in1)
  [status_bits] -> bus_create2/2(in2)
  bus_create2/1(bus_out) -> Delay4/1
  vacc0/2(dout_1_1) -> Slice1/1
  vacc0/3(dout_2_1) -> Slice11/1
  vacc1/2(dout_1_1) -> Slice17/1
  vacc1/3(dout_2_1) -> Slice23/1
  vacc2/2(dout_1_1) -> Slice32/1
  vacc2/3(dout_2_1) -> Slice33/1
  vacc3/2(dout_1_1) -> Slice36/1
  vacc3/3(dout_2_1) -> Slice37/1
  vacc0/4(dout_3_1) -> Slice12/1
  vacc0/5(dout_4_1) -> Slice16/1
  vacc2/4(dout_3_1) -> Slice34/1
  vacc2/5(dout_4_1) -> Slice35/1
  vacc3/4(dout_3_1) -> Slice38/1
  vacc3/5(dout_4_1) -> Slice39/1
  [sync_out0] -> vacc0/1(sync)
  [acc_len] -> vacc0/2(acc_len)
  [acc_len] -> vacc3/2(acc_len)
  [sync_out2] -> vacc2/1(sync)
  [sync_out3] -> vacc3/1(sync)
  [acc_len] -> vacc2/2(acc_len)
  vacc1/1(valid) -> [valid]
  vacc2/1(valid) -> Terminator4/1
  vacc3/1(valid) -> Terminator7/1
  vacc1/4(dout_3_1) -> Slice24/1
  vacc1/5(dout_4_1) -> Slice31/1
  [sync_out1] -> vacc1/1(sync)
  [acc_len] -> vacc1/2(acc_len)
  [xxout0] -> reinterp_vacc/1
  [yyout0] -> reinterp_vacc1/1
  [xyoutre0] -> reinterp_vacc2/1
  [xyoutim0] -> reinterp_vacc3/1
  [xxout1] -> reinterp_vacc4/1
  [yyout1] -> reinterp_vacc5/1
  [xyoutre1] -> reinterp_vacc6/1
  [xyoutim1] -> reinterp_vacc7/1
  [xxout2] -> reinterp_vacc8/1
  [yyout2] -> reinterp_vacc9/1
  [xyoutre2] -> reinterp_vacc10/1
  [xyoutim2] -> reinterp_vacc11/1
  [xxout3] -> reinterp_vacc12/1
  [yyout3] -> reinterp_vacc13/1
  [xyoutre3] -> reinterp_vacc14/1
  [xyoutim3] -> reinterp_vacc15/1
  vacc0/1(valid) -> Terminator1/1
  Delay2/1 -> Delay16/1, Delay1/1, Delay17/1, Delay8/1, Delay3/1
  Delay17/1 -> [sync_out0]
  Delay16/1 -> [sync_out1]
  Delay8/1 -> [sync_out2]
  Delay3/1 -> [sync_out3]
  Delay1/1 -> [sync_out]
  sg/1(sync_out) -> Subsytem/1(In1)
  Subsytem/1(Out1) -> [sync_gen_1]
  Subsytem/2(Out2) -> [sync_gen_0]
  sg/2(pps_out) -> Subsystem/1(In2)
  Subsystem/1(Out1) -> [master_rst1]
  Subsystem/2(Out2) -> [master_rst2]
  Subsystem/3(Out3) -> [master_rst3]
  Subsystem/4(Out4) -> [master_rst4]
  Slice1/1 -> [xx_vacc0]
  Slice11/1 -> [yy_vacc0]
  Slice12/1 -> [xy_vaccre0]
  Slice16/1 -> [xy_vaccim0]
  Slice17/1 -> [xx_vacc1]
  Slice23/1 -> [yy_vacc1]
  Slice24/1 -> [xy_vaccre1]
  Slice31/1 -> [xy_vaccim1]
  Slice32/1 -> [xx_vacc2]
  Slice33/1 -> [yy_vacc2]
  Slice34/1 -> [xy_vaccre2]
  Slice35/1 -> [xy_vaccim2]
  Slice36/1 -> [xx_vacc3]
  Slice37/1 -> [yy_vacc3]
  Slice38/1 -> [xy_vaccre3]
  Slice39/1 -> [xy_vaccim3]
  reinterp_vacc/1 -> vacc0/3(din_1_1)
  reinterp_vacc1/1 -> vacc0/4(din_2_1)
  reinterp_vacc2/1 -> vacc0/5(din_3_1)
  reinterp_vacc3/1 -> vacc0/6(din_4_1)
  reinterp_vacc4/1 -> vacc1/3(din_1_1)
  reinterp_vacc5/1 -> vacc1/4(din_2_1)
  reinterp_vacc6/1 -> vacc1/5(din_3_1)
  reinterp_vacc7/1 -> vacc1/6(din_4_1)
  reinterp_vacc8/1 -> vacc2/3(din_1_1)
  reinterp_vacc9/1 -> vacc2/4(din_2_1)
  reinterp_vacc10/1 -> vacc2/5(din_3_1)
  reinterp_vacc11/1 -> vacc2/6(din_4_1)
  reinterp_vacc12/1 -> vacc3/3(din_1_1)
  reinterp_vacc13/1 -> vacc3/4(din_2_1)
  reinterp_vacc14/1 -> vacc3/5(din_3_1)
  reinterp_vacc15/1 -> vacc3/6(din_4_1)
  Constant14/1 -> trig/1(sim_1)
  [spead_rst] -> sg/2(pps_en)
  ssg/1(statusbits) -> [status_bits]
  Subsystem1/1(Out1) -> bus_expand/1(bus_in), [adc_a]
  Subsystem2/1(Out1) -> bus_expand1/1(bus_in), [adc_b]
  asiaa_adc5g1/17(sync_out) -> Register44/1
  asiaa_adc5g2/17(sync_out) -> Terminator43/1
  asiaa_adc5g1/1(a0) -> Delay7/1
  asiaa_adc5g1/2(a1) -> Delay9/1
  asiaa_adc5g1/3(a2) -> Delay18/1
  asiaa_adc5g1/4(a3) -> Delay20/1
  asiaa_adc5g1/5(a4) -> Delay22/1
  asiaa_adc5g1/6(a5) -> Delay19/1
  asiaa_adc5g1/7(a6) -> Delay31/1
  asiaa_adc5g1/8(a7) -> Delay33/1
  asiaa_adc5g1/9(a8) -> Delay23/1
  asiaa_adc5g1/10(a9) -> Delay27/1
  asiaa_adc5g1/11(a10) -> Delay28/1
  asiaa_adc5g1/12(a11) -> Delay24/1
  asiaa_adc5g1/13(a12) -> Delay34/1
  asiaa_adc5g1/14(a13) -> Delay36/1
  asiaa_adc5g1/15(a14) -> Delay37/1
  asiaa_adc5g1/16(a15) -> Delay35/1
  asiaa_adc5g2/1(a0) -> Delay56/1
  asiaa_adc5g2/2(a1) -> Delay57/1
  asiaa_adc5g2/3(a2) -> Delay42/1
  asiaa_adc5g2/4(a3) -> Delay44/1
  asiaa_adc5g2/5(a4) -> Delay45/1
  asiaa_adc5g2/6(a5) -> Delay43/1
  asiaa_adc5g2/7(a6) -> Delay50/1
  asiaa_adc5g2/8(a7) -> Delay51/1
  asiaa_adc5g2/9(a8) -> Delay46/1
  asiaa_adc5g2/10(a9) -> Delay48/1
  asiaa_adc5g2/11(a10) -> Delay49/1
  asiaa_adc5g2/12(a11) -> Delay47/1
  asiaa_adc5g2/13(a12) -> Delay52/1
  asiaa_adc5g2/14(a13) -> Delay54/1
  asiaa_adc5g2/15(a14) -> Delay55/1
  asiaa_adc5g2/16(a15) -> Delay53/1
  Delay7/1 -> Subsystem1/1(In1)
  Delay9/1 -> Subsystem1/2(In2)
  Delay18/1 -> Subsystem1/3(In3)
  Delay20/1 -> Subsystem1/4(In4)
  Delay22/1 -> Subsystem1/5(In5)
  Delay19/1 -> Subsystem1/6(In6)
  Delay31/1 -> Subsystem1/7(In7)
  Delay33/1 -> Subsystem1/8(In8)
  Delay23/1 -> Subsystem1/9(In9)
  Delay27/1 -> Subsystem1/10(In10)
  Delay28/1 -> Subsystem1/11(In11)
  Delay24/1 -> Subsystem1/12(In12)
  Delay34/1 -> Subsystem1/13(In13)
  Delay36/1 -> Subsystem1/14(In14)
  Delay37/1 -> Subsystem1/15(In15)
  Delay35/1 -> Subsystem1/16(In16)
  Delay56/1 -> Subsystem2/1(In1)
  Delay57/1 -> Subsystem2/2(In2)
  Delay42/1 -> Subsystem2/3(In3)
  Delay44/1 -> Subsystem2/4(In4)
  Delay45/1 -> Subsystem2/5(In5)
  Delay43/1 -> Subsystem2/6(In6)
  Delay50/1 -> Subsystem2/7(In7)
  Delay51/1 -> Subsystem2/8(In8)
  Delay46/1 -> Subsystem2/9(In9)
  Delay48/1 -> Subsystem2/10(In10)
  Delay49/1 -> Subsystem2/11(In11)
  Delay47/1 -> Subsystem2/12(In12)
  Delay52/1 -> Subsystem2/13(In13)
  Delay54/1 -> Subsystem2/14(In14)
  Delay55/1 -> Subsystem2/15(In15)
  Delay53/1 -> Subsystem2/16(In16)
  [sync_gen_1] -> pfbfirr_15stages1/1
  [sync_gen_0] -> pfbfirr_15stages/1
  Delay5/1 -> fftwbr_15stages/2
  pfbfirr_15stages1/2 -> fftwbr_15stages/3
  pfbfirr_15stages1/3 -> fftwbr_15stages/4
  pfbfirr_15stages1/4 -> fftwbr_15stages/5
  pfbfirr_15stages1/5 -> fftwbr_15stages/6
  pfbfirr_15stages1/6 -> fftwbr_15stages/7
  pfbfirr_15stages1/7 -> fftwbr_15stages/8
  pfbfirr_15stages1/8 -> fftwbr_15stages/9
  pfbfirr_15stages1/9 -> fftwbr_15stages/10
  pfbfirr_15stages1/10 -> fftwbr_15stages/11
  pfbfirr_15stages1/11 -> fftwbr_15stages/12
  pfbfirr_15stages1/12 -> fftwbr_15stages/13
  pfbfirr_15stages1/13 -> fftwbr_15stages/14
  pfbfirr_15stages1/14 -> fftwbr_15stages/15
  pfbfirr_15stages1/15 -> fftwbr_15stages/16
  pfbfirr_15stages1/16 -> fftwbr_15stages/17
  pfbfirr_15stages1/17 -> fftwbr_15stages/18
  pfbfirr_15stages/2 -> fftwbr_15stages1/3
  pfbfirr_15stages/3 -> fftwbr_15stages1/4
  pfbfirr_15stages/4 -> fftwbr_15stages1/5
  pfbfirr_15stages/5 -> fftwbr_15stages1/6
  pfbfirr_15stages/6 -> fftwbr_15stages1/7
  pfbfirr_15stages/7 -> fftwbr_15stages1/8
  pfbfirr_15stages/8 -> fftwbr_15stages1/9
  pfbfirr_15stages/9 -> fftwbr_15stages1/10
  pfbfirr_15stages/10 -> fftwbr_15stages1/11
  pfbfirr_15stages/11 -> fftwbr_15stages1/12
  pfbfirr_15stages/12 -> fftwbr_15stages1/13
  pfbfirr_15stages/13 -> fftwbr_15stages1/14
  pfbfirr_15stages/14 -> fftwbr_15stages1/15
  pfbfirr_15stages/15 -> fftwbr_15stages1/16
  pfbfirr_15stages/16 -> fftwbr_15stages1/17
  pfbfirr_15stages/17 -> fftwbr_15stages1/18
  Delay6/1 -> fftwbr_15stages1/2
  fftwbr_15stages/1 -> Register9/1
  Register4/1 -> [xout4]
  Register5/1 -> [xout5]
  Register3/1 -> [xout6]
  Register6/1 -> [xout7]
  fftwbr_15stages/8 -> Register3/1
  fftwbr_15stages/9 -> Register6/1
  fftwbr_15stages/7 -> Register5/1
  fftwbr_15stages/6 -> Register4/1
  fftwbr_15stages/5 -> Register2/1
  fftwbr_15stages/4 -> Register1/1
  fftwbr_15stages/3 -> Register11/1
  fftwbr_15stages/2 -> Register10/1
  fftwbr_15stages1/1 -> Terminator2/1
  Register15/1 -> [yout5]
  Register7/1 -> [yout6]
  Register8/1 -> [yout7]
  fftwbr_15stages1/2 -> Register48/1
  fftwbr_15stages1/3 -> Register49/1
  fftwbr_15stages1/4 -> Register12/1
  Register14/1 -> [yout4]
  [xout4] -> Stokes/9(x4)
  [yout4] -> Stokes/10(y4)
  [xout5] -> Stokes/11(x5)
  [yout5] -> Stokes/12(y5)
  [xout6] -> Stokes/13(x6)
  [yout6] -> Stokes/14(y6)
  [xout7] -> Stokes/15(x7)
  [yout7] -> Stokes/16(y7)
  pfbfirr_15stages1/1 -> fftwbr_15stages/1
  [yout3] -> Stokes/8(y3)
  [xout3] -> Stokes/7(x3)
  [yout2] -> Stokes/6(y2)
  [xout2] -> Stokes/5(x2)
  [yout1] -> Stokes/4(y1)
  [xout1] -> Stokes/3(x1)
  [yout0] -> Stokes/2(y0)
  [xout0] -> Stokes/1(x0)
  Slice59/1 -> [yyout4]
  Slice44/1 -> [xyoutre4]
  Slice47/1 -> [xyoutim4]
  Slice48/1 -> [xxout5]
  Slice49/1 -> [yyout5]
  Slice50/1 -> [xyoutre5]
  Slice51/1 -> [xyoutim5]
  Slice56/1 -> [xxout6]
  Slice57/1 -> [yyout6]
  Slice45/1 -> [xyoutre6]
  Slice46/1 -> [xyoutim6]
  Slice52/1 -> [xxout7]
  Slice53/1 -> [yyout7]
  Slice54/1 -> [xyoutre7]
  Slice55/1 -> [xyoutim7]
  Slice58/1 -> [xxout4]
  Stokes/1(x0x0*) -> Slice5/1
  Stokes/2(y0y0*) -> Slice6/1
  Stokes/3(x0y0*_re) -> Slice13/1
  Stokes/4(x0y0*_im) -> Slice18/1
  Stokes/5(x1x1*) -> Slice19/1
  Stokes/6(y1y1*) -> Slice20/1
  Stokes/7(x1y1*_re) -> Slice21/1
  Stokes/8(x1y1*_im) -> Slice22/1
  Stokes/9(x2x2*) -> Slice29/1
  Stokes/10(y2y2*) -> Slice30/1
  Stokes/11(x2y2*_re) -> Slice14/1
  Stokes/12(x2y2*_im) -> Slice15/1
  Stokes/13(x3x3*) -> Slice25/1
  Stokes/14(y3y3*) -> Slice26/1
  Stokes/15(x3y3*_re) -> Slice27/1
  Stokes/16(x3y3*_im) -> Slice28/1
  Stokes/17(x4x4*) -> Slice58/1
  Stokes/18(y4y4*) -> Slice59/1
  Stokes/19(x4y4*_re) -> Slice44/1
  Stokes/20(x4y4*_im) -> Slice47/1
  Stokes/21(x5x5*) -> Slice48/1
  Stokes/22(y5y5*) -> Slice49/1
  Stokes/23(x5y5*_re) -> Slice50/1
  Stokes/24(x5y5*_im) -> Slice51/1
  Stokes/25(x6x6*) -> Slice56/1
  Stokes/26(y6y6*) -> Slice57/1
  Stokes/27(x6y6*_re) -> Slice45/1
  Stokes/28(x6y6*_im) -> Slice46/1
  Stokes/29(x7x7*) -> Slice52/1
  Stokes/30(y7y7*) -> Slice53/1
  Stokes/31(x7y7*_re) -> Slice54/1
  Stokes/32(x7y7*_im) -> Slice55/1
  vacc4/2(dout_1_1) -> Slice60/1
  vacc4/3(dout_2_1) -> Slice61/1
  vacc5/2(dout_1_1) -> Slice64/1
  vacc5/3(dout_2_1) -> Slice65/1
  vacc4/4(dout_3_1) -> Slice62/1
  vacc4/5(dout_4_1) -> Slice63/1
  vacc5/4(dout_3_1) -> Slice66/1
  vacc5/5(dout_4_1) -> Slice67/1
  [acc_len] -> vacc5/2(acc_len)
  [sync_out2] -> vacc4/1(sync)
  [sync_out3] -> vacc5/1(sync)
  [acc_len] -> vacc4/2(acc_len)
  vacc4/1(valid) -> Terminator14/1
  vacc5/1(valid) -> Terminator18/1
  [xxout6] -> reinterp_vacc22/1
  [yyout6] -> reinterp_vacc23/1
  [xyoutre6] -> reinterp_vacc16/1
  [xyoutim6] -> reinterp_vacc17/1
  [xxout7] -> reinterp_vacc18/1
  [yyout7] -> reinterp_vacc19/1
  [xyoutre7] -> reinterp_vacc20/1
  [xyoutim7] -> reinterp_vacc21/1
  Slice60/1 -> [xx_vacc6]
  Slice61/1 -> [yy_vacc6]
  Slice62/1 -> [xy_vaccre6]
  Slice63/1 -> [xy_vaccim6]
  Slice64/1 -> [xx_vacc7]
  Slice65/1 -> [yy_vacc7]
  Slice66/1 -> [xy_vaccre7]
  Slice67/1 -> [xy_vaccim7]
  reinterp_vacc22/1 -> vacc4/3(din_1_1)
  reinterp_vacc23/1 -> vacc4/4(din_2_1)
  reinterp_vacc16/1 -> vacc4/5(din_3_1)
  reinterp_vacc17/1 -> vacc4/6(din_4_1)
  reinterp_vacc18/1 -> vacc5/3(din_1_1)
  reinterp_vacc19/1 -> vacc5/4(din_2_1)
  reinterp_vacc20/1 -> vacc5/5(din_3_1)
  reinterp_vacc21/1 -> vacc5/6(din_4_1)
  vacc6/2(dout_1_1) -> Slice68/1
  vacc6/3(dout_2_1) -> Slice69/1
  vacc7/2(dout_1_1) -> Slice72/1
  vacc7/3(dout_2_1) -> Slice73/1
  vacc6/4(dout_3_1) -> Slice70/1
  vacc6/5(dout_4_1) -> Slice71/1
  [sync_out0] -> vacc6/1(sync)
  [acc_len] -> vacc6/2(acc_len)
  vacc7/1(valid) -> Terminator20/1
  vacc7/4(dout_3_1) -> Slice74/1
  vacc7/5(dout_4_1) -> Slice75/1
  [sync_out1] -> vacc7/1(sync)
  [acc_len] -> vacc7/2(acc_len)
  [xxout4] -> reinterp_vacc24/1
  [yyout4] -> reinterp_vacc25/1
  [xyoutre4] -> reinterp_vacc26/1
  [xyoutim4] -> reinterp_vacc27/1
  [xxout5] -> reinterp_vacc28/1
  [yyout5] -> reinterp_vacc29/1
  [xyoutre5] -> reinterp_vacc30/1
  [xyoutim5] -> reinterp_vacc31/1
  vacc6/1(valid) -> Terminator19/1
  Slice68/1 -> [xx_vacc4]
  Slice69/1 -> [yy_vacc4]
  Slice70/1 -> [xy_vaccre4]
  Slice71/1 -> [xy_vaccim4]
  Slice72/1 -> [xx_vacc5]
  Slice73/1 -> [yy_vacc5]
  Slice74/1 -> [xy_vaccre5]
  Slice75/1 -> [xy_vaccim5]
  reinterp_vacc24/1 -> vacc6/3(din_1_1)
  reinterp_vacc25/1 -> vacc6/4(din_2_1)
  reinterp_vacc26/1 -> vacc6/5(din_3_1)
  reinterp_vacc27/1 -> vacc6/6(din_4_1)
  reinterp_vacc28/1 -> vacc7/3(din_1_1)
  reinterp_vacc29/1 -> vacc7/4(din_2_1)
  reinterp_vacc30/1 -> vacc7/5(din_3_1)
  reinterp_vacc31/1 -> vacc7/6(din_4_1)
  [xy_vaccre7] -> cram4/1(In1)
  [xy_vaccim7] -> cram4/2(In2)
  [xx_vacc7] -> cram4/3(In3)
  [yy_vacc7] -> cram4/4(In4)
  [xy_vaccre6] -> cram4/5(In5)
  [xy_vaccim6] -> cram4/6(In6)
  [xx_vacc6] -> cram4/7(In7)
  [yy_vacc6] -> cram4/8(In8)
  [xy_vaccre5] -> cram4/9(In9)
  [xy_vaccim5] -> cram4/10(In10)
  [xx_vacc5] -> cram4/11(In11)
  [yy_vacc5] -> cram4/12(In12)
  [xy_vaccre4] -> cram4/13(In13)
  [xy_vaccim4] -> cram4/14(In14)
  [xx_vacc4] -> cram4/15(In15)
  [yy_vacc4] -> cram4/16(In16)
  [xy_vaccre3] -> cram4/17(In17)
  [xy_vaccim3] -> cram4/18(In18)
  [xx_vacc3] -> cram4/19(In19)
  [yy_vacc3] -> cram4/20(In20)
  [xy_vaccre2] -> cram4/21(In21)
  [xy_vaccim2] -> cram4/22(In22)
  [xx_vacc2] -> cram4/23(In23)
  [yy_vacc2] -> cram4/24(In24)
  [xy_vaccre1] -> cram4/25(In25)
  [xy_vaccim1] -> cram4/26(In26)
  [xx_vacc1] -> cram4/27(In27)
  [yy_vacc1] -> cram4/28(In28)
  [xy_vaccre0] -> cram4/29(In29)
  [xy_vaccim0] -> cram4/30(In30)
  [xx_vacc0] -> cram4/31(In31)
  [yy_vacc0] -> cram4/32(In32)
  bus_expand1/1(msb_out16) -> pfbfirr_15stages/2
  bus_expand1/2(out15) -> pfbfirr_15stages/3
  bus_expand1/3(out14) -> pfbfirr_15stages/4
  bus_expand1/4(out13) -> pfbfirr_15stages/5
  bus_expand1/5(out12) -> pfbfirr_15stages/6
  bus_expand1/6(out11) -> pfbfirr_15stages/7
  bus_expand1/7(out10) -> pfbfirr_15stages/8
  bus_expand1/8(out9) -> pfbfirr_15stages/9
  bus_expand1/9(out8) -> pfbfirr_15stages/10
  bus_expand1/10(out7) -> pfbfirr_15stages/11
  bus_expand1/11(out6) -> pfbfirr_15stages/12
  bus_expand1/12(out5) -> pfbfirr_15stages/13
  bus_expand1/13(out4) -> pfbfirr_15stages/14
  bus_expand1/14(out3) -> pfbfirr_15stages/15
  bus_expand1/15(out2) -> pfbfirr_15stages/16
  bus_expand1/16(lsb_out1) -> pfbfirr_15stages/17
  trig/1(in_reg) -> Slice/1
  Slice/1 -> adcsnap1/3(trig), adcsnap0/3(trig)
  [adc_b] -> adcsnap1/1(din)
  [adc_a] -> adcsnap0/1(din)
  Constant17/1 -> adcsnap1/2(we)
  Constant13/1 -> adcsnap0/2(we)
  Slice40/1 -> Delay38/1
  Delay38/1 -> nspec/1(out_reg)
  [spec_cntr] -> Slice40/1
  bus_create/1(bus_out) -> Delay39/1
  Delay39/1 -> status/1(out_reg)
  [data_valid] -> bus_create/1(in1)
  [eoh] -> bus_create/2(in2)
  [eof] -> bus_create/3(in3)
  [spead_st] -> bus_create/4(in4)
  [data_valid_spead] -> bus_create/5(in5)
  [reshape_state] -> bus_create/6(in6)
  [data_enable] -> bus_create/7(in7)
  [spead_rst] -> bus_create/8(in8)
  [master_rst1] -> bus_create/9(in9)
  [tge_rst] -> bus_create/10(in10)
  [valid] -> bus_create/11(in11)
  [txovf] -> bus_create/12(in12)
  [xxout0] -> stokesout/1(din)
  [sync_out1] -> stokesout/2(we), stokesout/3(trig)
  [master_rst2] -> Register/1
  Register/1 -> ssg/1(reset)
  [spec_tick] -> ssg/2(spec_tick)
  fftwbr_15stages1/10 -> Terminator30/1
  fftwbr_15stages1/9 -> Register8/1
  fftwbr_15stages1/8 -> Register7/1
  fftwbr_15stages1/7 -> Register15/1
  fftwbr_15stages1/6 -> Register14/1
  fftwbr_15stages1/5 -> Register13/1
  [master_rst1] -> pkt_cntr1/1
  [eof] -> pkt_cntr1/2
  pkt_cntr1/1 -> Delay59/1
  Delay59/1 -> npkt/1(out_reg)
  edge_detect5/1(out) -> [adc_sync]
  edge_detect4/1(out) -> Delay61/1
  Delay60/1 -> Logical2/2
  Delay61/1 -> reshaper/1(rst)
  [time_cntr] -> timesnap/1(din)
  edge_detect/1(out) -> timesnap/2(we)
  [master_rst1] -> timesnap/3(trig)
  Mux/1 -> edge_detect/1(in)
  [sync_out0] -> Mux/2
  [valid] -> Mux/3
  [data_valid_spead] -> Mux/5
  [data_valid] -> Mux/4
  Convert1/1 -> Mux/1
  Constant1/1 -> timesel/1(sim_1)
  timesel/1(in_reg) -> Convert1/1
  fftshift/1(in_reg) -> [fftshift]
  Constant2/1 -> fftshift/1(sim_1)
  pfbfirr_15stages/1 -> fftwbr_15stages1/1
  bus_expand/1(msb_out16) -> pfbfirr_15stages1/2
  bus_expand/2(out15) -> pfbfirr_15stages1/3
  bus_expand/3(out14) -> pfbfirr_15stages1/4
  bus_expand/4(out13) -> pfbfirr_15stages1/5
  bus_expand/5(out12) -> pfbfirr_15stages1/6
  bus_expand/6(out11) -> pfbfirr_15stages1/7
  bus_expand/7(out10) -> pfbfirr_15stages1/8
  bus_expand/8(out9) -> pfbfirr_15stages1/9
  bus_expand/9(out8) -> pfbfirr_15stages1/10
  bus_expand/10(out7) -> pfbfirr_15stages1/11
  bus_expand/11(out6) -> pfbfirr_15stages1/12
  bus_expand/12(out5) -> pfbfirr_15stages1/13
  bus_expand/13(out4) -> pfbfirr_15stages1/14
  bus_expand/14(out3) -> pfbfirr_15stages1/15
  bus_expand/15(out2) -> pfbfirr_15stages1/16
  bus_expand/16(lsb_out1) -> pfbfirr_15stages1/17
  Counter2/1 -> Relational2/1
  Constant4/1 -> Relational2/2
  Relational2/1 -> Delay/1
  edge_detect6/1(out) -> Delay58/1
  Delay/1 -> Logical1/2
  Delay58/1 -> Logical1/1
  Slice41/1 -> Delay40/1
  Logical1/1 -> rshpout/3(trig)
  Delay40/1 -> rshpout/1(din)
  Delay41/1 -> rshpout/2(we)
